simulink model "DualStreamSSR"  (R2020b)
(part 3 of 5)

  filter30 : ModelComposer/AIE Class Kernel  KernelAllAttrs=|  PortNames={'sin1'; 'sin2'; 'cout'}  PortSerializedTypes={'{Q2{P{Tinput_stream{1{t{Scint16}}}}}}'; '{Q2{P{Tinput_stream{1{t{Scint16}}}}}}'; '{P{Toutput_stream{1{t{Scacc48_t}}}}}'}  PortWindowSizes={0.000000000000000000e+00; 0.000000000000000000e+00; 0.000000000000000000e+00}  PortWindowMargins={0.000000000000000000e+00; 0.000000000000000000e+00; 0.000000000000000000e+00}  PortSynchronicities={'auto'; 'auto'; 'auto'}  PortSignalSizes={0.000000000000000000e+00; 0.000000000000000000e+00; 8.000000000000000000e+00}  ClassTemplateSpecKind=implicit  ClassTemplateParamNames={'NSamples'; 'ShiftAcc'; 'DiscardSample'; 'SwapRead'}  ClassTemplateParamKinds={'nontype'; 'nontype'; 'nontype'; 'nontype'}  ClassTemplateParamTypes={'int'; 'int'; 'bool'; 'bool'}  ClassTemplateParamValues={'512', '15', '0', '0'}  ClassCtorParamNames={'taps'}  ClassCtorParamSerializedTypes={'{R{Q1{C{Scint16}4}}}'}  ClassCtorParamValues={'[-121-233i 237-96i 1454+497i 14+121i]'}  ClassIndex=1  ClassCtorIndex=1  ClassTabVisible=on  ClassTemplateParamsVisible=on  ClassCtorDeclVisible=on  ClassCtorParamsVisible=on  FunctionTabVisible=on  FunctionDecl=|  PortAttrs={ 'input', 'sin1', 'input_stream_cint16 * restrict', '', '', '', ''; 'input', 'sin2', 'input_stream_cint16 * restrict', '', '', '', ''; 'output', 'cout', 'output_stream< cacc48_t > *', '', '', '', 'OUTPUT_SIZE' }  PortAttrsEnables={'off', 'off', 'off', 'off', 'off', 'off', 'off';'off', 'off', 'off', 'off', 'off', 'off', 'off';'off', 'off', 'off', 'off', 'off', 'off', 'on'}  SampleTime=-1  ClassDeclTypeOptions=|  ClassDecl=|  ClassTemplateParams={ 'NSamples', 'int', 'BURST_LENGTH'; 'ShiftAcc', 'int', 'SHIFT_ACC'; 'DiscardSample', 'bool', 'FALSE'; 'SwapRead', 'bool', 'FALSE' }  ClassTemplateParamsEnables={'off', 'off', 'on';'off', 'off', 'on';'off', 'off', 'on';'off', 'off', 'on'}  ClassCtorDeclTypeOptions=C[1 1]@t51@FIR_MultiKernel_cout(cint16 const ( & taps ) [ 4 ])  ClassCtorDecl=FIR_MultiKernel_cout(cint16 const ( & taps ) [ 4 ])  ClassCtorParams={ 'taps', 'cint16 const ( &) [ 4 ]', 'phi_4' }  KernelHeaderFile=FirDoubleStream.h  KernelClassName=DoubleStream::FIR_MultiKernel_cout  KernelFunction=filter  KernelSourceFile=FirDoubleStream.cpp  KernelSearchPaths={'$SRC/aie_kernels'}  PreProcOptions={}  CoreRuntimeRatio=0.9  KernelLocSpec=off  ColRowLocation=[0 0]  blockJsonConstraints="[{\"type\":\"constraint\",\"constraintType\":\"coreUtilization\",\"sid\":\"49\",\"lhs\":{\"type\":\"runtimeRatio\",\"args\":{\"type\":\"kernel\",\"name\":\"DualStreamSSR_1/Subsystem/filter30\",\"sid\":\"49\"}},\"rhs\":{\"type\":\"evaluable\",\"expr\":\"0.9\",\"value\":0.9},\"equality\":true},{\"type\":\"constraint\",\"constraintType\":\"location_kernel\",\"sid\":\"49\",\"lhs\":{\"type\":\"location\",\"templParam\":\"kernel\",\"args\":{\"type\":\"kernel\",\"name\":\"DualStreamSSR_1/Subsystem/filter30\",\"sid\":\"49\"}},\"rhs\":{\"type\":\"tile\",\"args\":[{\"type\":\"evaluable\",\"expr\":\"30\",\"value\":30},{\"type\":\"evaluable\",\"expr\":\"3\",\"value\":3}]},\"equality\":true}]"  deprecateConstraints=1
      KernelAllAttrs=|
      | s[12;12;9;9;19;14;21;23;24;21;12;24;26;26;26;27;28;9;21;23;23;23;24;25;14;19;19;29]@FunctionNameDeclFileNamePortNamesPortTypesPortSerializedTypesPortDirectionsPortWindowSizeEnablesPortWindowMarginEnablesPortSynchronicityEnablesPortSignalSizeEnablesFunctionDeclFunctionTemplateSpecKindFunctionTemplateParamNamesFunctionTemplateParamKindsFunctionTemplateParamTypesFunctionTemplateParamValuesFunctionTemplateParamEnablesClassDeclClassTemplateSpecKindClassTemplateParamNamesClassTemplateParamKindsClassTemplateParamTypesClassTemplateParamValuesClassTemplateParamEnablesClassCtorDeclsClassCtorParamNamesClassCtorParamTypesClassCtorParamSerializedTypes[1 1]@C[28 1]@t6@filtert42@../../../aie/aie_kernels/FirDoubleStream.hC[3 1]@t4@sin1t4@sin2t4@coutC[3 1]@t30@input_stream_cint16 * restrictt30@input_stream_cint16 * restrictt27@output_stream< cacc48_t > *C[3 1]@t37@{Q2{P{Tinput_stream{1{t{Scint16}}}}}}t37@{Q2{P{Tinput_stream{1{t{Scint16}}}}}}t36@{P{Toutput_stream{1{t{Scacc48_t}}}}}C[3 1]@t5@inputt5@inputt6@outputC[3 1]@l0@l0@l0@C[3 1]@l0@l0@l0@C[3 1]@l0@l0@l0@C[3 1]@l0@l0@l1@t246@namespace DoubleStream {
      | template < int NSamples, int ShiftAcc, bool DiscardSample, bool SwapRead > 
      | void FIR_MultiKernel_cout::
      | filter(input_stream_cint16 * restrict sin1, input_stream_cint16 * restrict sin2, output_stream< cacc48_t > * cout);
      | }t4@nonee[0 1]@e[0 1]@e[0 1]@e[0 1]@e[0 1]@t129@namespace DoubleStream {
      | template < int NSamples, int ShiftAcc, bool DiscardSample, bool SwapRead > class FIR_MultiKernel_cout;
      | }t8@implicitC[4 1]@t8@NSamplest8@ShiftAcct13@DiscardSamplet8@SwapReadC[4 1]@t7@nontypet7@nontypet7@nontypet7@nontypeC[4 1]@t3@intt3@intt4@boolt4@boolC[4 1]@nnnnC[4 1]@l1@l1@l1@l1@C[1 1]@t51@FIR_MultiKernel_cout(cint16 const ( & taps ) [ 4 ])C[1 1]@C[1 1]@t4@tapsC[1 1]@C[1 1]@t23@cint16 const ( &) [ 4 ]C[1 1]@C[1 1]@t20@{R{Q1{C{Scint16}4}}}
      FunctionDecl=|
      | namespace DoubleStream {
      | template < int NSamples, int ShiftAcc, bool DiscardSample, bool SwapRead > 
      | void FIR_MultiKernel_cout::
      | filter(input_stream_cint16 * restrict sin1, input_stream_cint16 * restrict sin2, output_stream< cacc48_t > * cout);
      | }
      ClassDeclTypeOptions=|
      | C[1 1]@t129@namespace DoubleStream {
      | template < int NSamples, int ShiftAcc, bool DiscardSample, bool SwapRead > class FIR_MultiKernel_cout;
      | }
      ClassDecl=|
      | namespace DoubleStream {
      | template < int NSamples, int ShiftAcc, bool DiscardSample, bool SwapRead > class FIR_MultiKernel_cout;
      | }
  filter31 : ModelComposer/AIE Class Kernel  KernelAllAttrs=|  PortNames={'sin1'; 'sin2'; 'cin'; 'cout'}  PortSerializedTypes={'{Q2{P{Tinput_stream{1{t{Scint16}}}}}}'; '{Q2{P{Tinput_stream{1{t{Scint16}}}}}}'; '{P{Tinput_stream{1{t{Scacc48_t}}}}}'; '{P{Toutput_stream{1{t{Scacc48_t}}}}}'}  PortWindowSizes={0.000000000000000000e+00; 0.000000000000000000e+00; 0.000000000000000000e+00; 0.000000000000000000e+00}  PortWindowMargins={0.000000000000000000e+00; 0.000000000000000000e+00; 0.000000000000000000e+00; 0.000000000000000000e+00}  PortSynchronicities={'auto'; 'auto'; 'auto'; 'auto'}  PortSignalSizes={0.000000000000000000e+00; 0.000000000000000000e+00; 0.000000000000000000e+00; 8.000000000000000000e+00}  ClassTemplateSpecKind=implicit  ClassTemplateParamNames={'NSamples'; 'ShiftAcc'; 'DiscardSample'; 'SwapRead'}  ClassTemplateParamKinds={'nontype'; 'nontype'; 'nontype'; 'nontype'}  ClassTemplateParamTypes={'int'; 'int'; 'bool'; 'bool'}  ClassTemplateParamValues={'512', '15', '0', '0'}  ClassCtorParamNames={'taps'}  ClassCtorParamSerializedTypes={'{R{Q1{C{Scint16}4}}}'}  ClassCtorParamValues={'[14-121i 1454-497i 237+96i -121+233i]'}  ClassIndex=1  ClassCtorIndex=1  ClassTabVisible=on  ClassTemplateParamsVisible=on  ClassCtorDeclVisible=on  ClassCtorParamsVisible=on  FunctionTabVisible=on  FunctionDecl=|  PortAttrs={ 'input', 'sin1', 'input_stream_cint16 * restrict', '', '', '', ''; 'input', 'sin2', 'input_stream_cint16 * restrict', '', '', '', ''; 'input', 'cin', 'input_stream< cacc48_t > *', '', '', '', ''; 'output', 'cout', 'output_stream< cacc48_t > *', '', '', '', 'OUTPUT_SIZE' }  PortAttrsEnables={'off', 'off', 'off', 'off', 'off', 'off', 'off';'off', 'off', 'off', 'off', 'off', 'off', 'off';'off', 'off', 'off', 'off', 'off', 'off', 'off';'off', 'off', 'off', 'off', 'off', 'off', 'on'}  SampleTime=-1  ClassDeclTypeOptions=|  ClassDecl=|  ClassTemplateParams={ 'NSamples', 'int', 'BURST_LENGTH'; 'ShiftAcc', 'int', 'SHIFT_ACC'; 'DiscardSample', 'bool', 'FALSE'; 'SwapRead', 'bool', 'FALSE' }  ClassTemplateParamsEnables={'off', 'off', 'on';'off', 'off', 'on';'off', 'off', 'on';'off', 'off', 'on'}  ClassCtorDeclTypeOptions=C[1 1]@t54@FIR_MultiKernel_cincout(cint16 const ( & taps ) [ 4 ])  ClassCtorDecl=FIR_MultiKernel_cincout(cint16 const ( & taps ) [ 4 ])  ClassCtorParams={ 'taps', 'cint16 const ( &) [ 4 ]', 'phi_3' }  KernelHeaderFile=FirDoubleStream.h  KernelClassName=DoubleStream::FIR_MultiKernel_cincout  KernelFunction=filter  KernelSourceFile=FirDoubleStream.cpp  KernelSearchPaths={'$SRC/aie_kernels'}  PreProcOptions={}  CoreRuntimeRatio=0.9  KernelLocSpec=off  ColRowLocation=[0 0]  blockJsonConstraints="{\"type\":\"constraint\",\"constraintType\":\"coreUtilization\",\"sid\":\"41\",\"lhs\":{\"type\":\"runtimeRatio\",\"args\":{\"type\":\"kernel\",\"name\":\"DualStreamSSR_1/Subsystem/filter22\",\"sid\":\"41\"}},\"rhs\":{\"type\":\"evaluable\",\"expr\":\"0.9\",\"value\":0.9},\"equality\":true}"  deprecateConstraints=1
      KernelAllAttrs=|
      | s[12;12;9;9;19;14;21;23;24;21;12;24;26;26;26;27;28;9;21;23;23;23;24;25;14;19;19;29]@FunctionNameDeclFileNamePortNamesPortTypesPortSerializedTypesPortDirectionsPortWindowSizeEnablesPortWindowMarginEnablesPortSynchronicityEnablesPortSignalSizeEnablesFunctionDeclFunctionTemplateSpecKindFunctionTemplateParamNamesFunctionTemplateParamKindsFunctionTemplateParamTypesFunctionTemplateParamValuesFunctionTemplateParamEnablesClassDeclClassTemplateSpecKindClassTemplateParamNamesClassTemplateParamKindsClassTemplateParamTypesClassTemplateParamValuesClassTemplateParamEnablesClassCtorDeclsClassCtorParamNamesClassCtorParamTypesClassCtorParamSerializedTypes[1 1]@C[28 1]@t6@filtert42@../../../aie/aie_kernels/FirDoubleStream.hC[4 1]@t4@sin1t4@sin2t3@cint4@coutC[4 1]@t30@input_stream_cint16 * restrictt30@input_stream_cint16 * restrictt26@input_stream< cacc48_t > *t27@output_stream< cacc48_t > *C[4 1]@t37@{Q2{P{Tinput_stream{1{t{Scint16}}}}}}t37@{Q2{P{Tinput_stream{1{t{Scint16}}}}}}t35@{P{Tinput_stream{1{t{Scacc48_t}}}}}t36@{P{Toutput_stream{1{t{Scacc48_t}}}}}C[4 1]@t5@inputt5@inputt5@inputt6@outputC[4 1]@l0@l0@l0@l0@C[4 1]@l0@l0@l0@l0@C[4 1]@l0@l0@l0@l0@C[4 1]@l0@l0@l0@l1@t281@namespace DoubleStream {
      | template < int NSamples, int ShiftAcc, bool DiscardSample, bool SwapRead > 
      | void FIR_MultiKernel_cincout::
      | filter(input_stream_cint16 * restrict sin1, input_stream_cint16 * restrict sin2, input_stream< cacc48_t > * cin, output_stream< cacc48_t > * cout);
      | }t4@nonee[0 1]@e[0 1]@e[0 1]@e[0 1]@e[0 1]@t132@namespace DoubleStream {
      | template < int NSamples, int ShiftAcc, bool DiscardSample, bool SwapRead > class FIR_MultiKernel_cincout;
      | }t8@implicitC[4 1]@t8@NSamplest8@ShiftAcct13@DiscardSamplet8@SwapReadC[4 1]@t7@nontypet7@nontypet7@nontypet7@nontypeC[4 1]@t3@intt3@intt4@boolt4@boolC[4 1]@nnnnC[4 1]@l1@l1@l1@l1@C[1 1]@t54@FIR_MultiKernel_cincout(cint16 const ( & taps ) [ 4 ])C[1 1]@C[1 1]@t4@tapsC[1 1]@C[1 1]@t23@cint16 const ( &) [ 4 ]C[1 1]@C[1 1]@t20@{R{Q1{C{Scint16}4}}}
      FunctionDecl=|
      | namespace DoubleStream {
      | template < int NSamples, int ShiftAcc, bool DiscardSample, bool SwapRead > 
      | void FIR_MultiKernel_cincout::
      | filter(input_stream_cint16 * restrict sin1, input_stream_cint16 * restrict sin2, input_stream< cacc48_t > * cin, output_stream< cacc48_t > * cout);
      | }
      ClassDeclTypeOptions=|
      | C[1 1]@t132@namespace DoubleStream {
      | template < int NSamples, int ShiftAcc, bool DiscardSample, bool SwapRead > class FIR_MultiKernel_cincout;
      | }
      ClassDecl=|
      | namespace DoubleStream {
      | template < int NSamples, int ShiftAcc, bool DiscardSample, bool SwapRead > class FIR_MultiKernel_cincout;
      | }
  filter32 : ModelComposer/AIE Class Kernel  KernelAllAttrs=|  PortNames={'sin1'; 'sin2'; 'cout'}  PortSerializedTypes={'{Q2{P{Tinput_stream{1{t{Scint16}}}}}}'; '{Q2{P{Tinput_stream{1{t{Scint16}}}}}}'; '{P{Toutput_stream{1{t{Scacc48_t}}}}}'}  PortWindowSizes={0.000000000000000000e+00; 0.000000000000000000e+00; 0.000000000000000000e+00}  PortWindowMargins={0.000000000000000000e+00; 0.000000000000000000e+00; 0.000000000000000000e+00}  PortSynchronicities={'auto'; 'auto'; 'auto'}  PortSignalSizes={0.000000000000000000e+00; 0.000000000000000000e+00; 8.000000000000000000e+00}  ClassTemplateSpecKind=implicit  ClassTemplateParamNames={'NSamples'; 'ShiftAcc'; 'DiscardSample'; 'SwapRead'}  ClassTemplateParamKinds={'nontype'; 'nontype'; 'nontype'; 'nontype'}  ClassTemplateParamTypes={'int'; 'int'; 'bool'; 'bool'}  ClassTemplateParamValues={'512', '15', '1', '0'}  ClassCtorParamNames={'taps'}  ClassCtorParamSerializedTypes={'{R{Q1{C{Scint16}4}}}'}  ClassCtorParamValues={'[-121-233i 237-96i 1454+497i 14+121i]'}  ClassIndex=1  ClassCtorIndex=1  ClassTabVisible=on  ClassTemplateParamsVisible=on  ClassCtorDeclVisible=on  ClassCtorParamsVisible=on  FunctionTabVisible=on  FunctionDecl=|  PortAttrs={ 'input', 'sin1', 'input_stream_cint16 * restrict', '', '', '', ''; 'input', 'sin2', 'input_stream_cint16 * restrict', '', '', '', ''; 'output', 'cout', 'output_stream< cacc48_t > *', '', '', '', 'OUTPUT_SIZE' }  PortAttrsEnables={'off', 'off', 'off', 'off', 'off', 'off', 'off';'off', 'off', 'off', 'off', 'off', 'off', 'off';'off', 'off', 'off', 'off', 'off', 'off', 'on'}  SampleTime=-1  ClassDeclTypeOptions=|  ClassDecl=|  ClassTemplateParams={ 'NSamples', 'int', 'BURST_LENGTH'; 'ShiftAcc', 'int', 'SHIFT_ACC'; 'DiscardSample', 'bool', 'TRUE'; 'SwapRead', 'bool', 'FALSE' }  ClassTemplateParamsEnables={'off', 'off', 'on';'off', 'off', 'on';'off', 'off', 'on';'off', 'off', 'on'}  ClassCtorDeclTypeOptions=C[1 1]@t51@FIR_MultiKernel_cout(cint16 const ( & taps ) [ 4 ])  ClassCtorDecl=FIR_MultiKernel_cout(cint16 const ( & taps ) [ 4 ])  ClassCtorParams={ 'taps', 'cint16 const ( &) [ 4 ]', 'phi_4' }  KernelHeaderFile=FirDoubleStream.h  KernelClassName=DoubleStream::FIR_MultiKernel_cout  KernelFunction=filter  KernelSourceFile=FirDoubleStream.cpp  KernelSearchPaths={'$SRC/aie_kernels'}  PreProcOptions={}  CoreRuntimeRatio=0.9  KernelLocSpec=off  ColRowLocation=[0 0]  blockJsonConstraints="[{\"type\":\"constraint\",\"constraintType\":\"coreUtilization\",\"sid\":\"51\",\"lhs\":{\"type\":\"runtimeRatio\",\"args\":{\"type\":\"kernel\",\"name\":\"DualStreamSSR_1/Subsystem/filter32\",\"sid\":\"51\"}},\"rhs\":{\"type\":\"evaluable\",\"expr\":\"0.9\",\"value\":0.9},\"equality\":true},{\"type\":\"constraint\",\"constraintType\":\"location_kernel\",\"sid\":\"51\",\"lhs\":{\"type\":\"location\",\"templParam\":\"kernel\",\"args\":{\"type\":\"kernel\",\"name\":\"DualStreamSSR_1/Subsystem/filter32\",\"sid\":\"51\"}},\"rhs\":{\"type\":\"tile\",\"args\":[{\"type\":\"evaluable\",\"expr\":\"23\",\"value\":23},{\"type\":\"evaluable\",\"expr\":\"4\",\"value\":4}]},\"equality\":true}]"  deprecateConstraints=1
      KernelAllAttrs=|
      | s[12;12;9;9;19;14;21;23;24;21;12;24;26;26;26;27;28;9;21;23;23;23;24;25;14;19;19;29]@FunctionNameDeclFileNamePortNamesPortTypesPortSerializedTypesPortDirectionsPortWindowSizeEnablesPortWindowMarginEnablesPortSynchronicityEnablesPortSignalSizeEnablesFunctionDeclFunctionTemplateSpecKindFunctionTemplateParamNamesFunctionTemplateParamKindsFunctionTemplateParamTypesFunctionTemplateParamValuesFunctionTemplateParamEnablesClassDeclClassTemplateSpecKindClassTemplateParamNamesClassTemplateParamKindsClassTemplateParamTypesClassTemplateParamValuesClassTemplateParamEnablesClassCtorDeclsClassCtorParamNamesClassCtorParamTypesClassCtorParamSerializedTypes[1 1]@C[28 1]@t6@filtert42@../../../aie/aie_kernels/FirDoubleStream.hC[3 1]@t4@sin1t4@sin2t4@coutC[3 1]@t30@input_stream_cint16 * restrictt30@input_stream_cint16 * restrictt27@output_stream< cacc48_t > *C[3 1]@t37@{Q2{P{Tinput_stream{1{t{Scint16}}}}}}t37@{Q2{P{Tinput_stream{1{t{Scint16}}}}}}t36@{P{Toutput_stream{1{t{Scacc48_t}}}}}C[3 1]@t5@inputt5@inputt6@outputC[3 1]@l0@l0@l0@C[3 1]@l0@l0@l0@C[3 1]@l0@l0@l0@C[3 1]@l0@l0@l1@t246@namespace DoubleStream {
      | template < int NSamples, int ShiftAcc, bool DiscardSample, bool SwapRead > 
      | void FIR_MultiKernel_cout::
      | filter(input_stream_cint16 * restrict sin1, input_stream_cint16 * restrict sin2, output_stream< cacc48_t > * cout);
      | }t4@nonee[0 1]@e[0 1]@e[0 1]@e[0 1]@e[0 1]@t129@namespace DoubleStream {
      | template < int NSamples, int ShiftAcc, bool DiscardSample, bool SwapRead > class FIR_MultiKernel_cout;
      | }t8@implicitC[4 1]@t8@NSamplest8@ShiftAcct13@DiscardSamplet8@SwapReadC[4 1]@t7@nontypet7@nontypet7@nontypet7@nontypeC[4 1]@t3@intt3@intt4@boolt4@boolC[4 1]@nnnnC[4 1]@l1@l1@l1@l1@C[1 1]@t51@FIR_MultiKernel_cout(cint16 const ( & taps ) [ 4 ])C[1 1]@C[1 1]@t4@tapsC[1 1]@C[1 1]@t23@cint16 const ( &) [ 4 ]C[1 1]@C[1 1]@t20@{R{Q1{C{Scint16}4}}}
      FunctionDecl=|
      | namespace DoubleStream {
      | template < int NSamples, int ShiftAcc, bool DiscardSample, bool SwapRead > 
      | void FIR_MultiKernel_cout::
      | filter(input_stream_cint16 * restrict sin1, input_stream_cint16 * restrict sin2, output_stream< cacc48_t > * cout);
      | }
      ClassDeclTypeOptions=|
      | C[1 1]@t129@namespace DoubleStream {
      | template < int NSamples, int ShiftAcc, bool DiscardSample, bool SwapRead > class FIR_MultiKernel_cout;
      | }
      ClassDecl=|
      | namespace DoubleStream {
      | template < int NSamples, int ShiftAcc, bool DiscardSample, bool SwapRead > class FIR_MultiKernel_cout;
      | }
  filter33 : ModelComposer/AIE Class Kernel  KernelAllAttrs=|  PortNames={'sin1'; 'sin2'; 'cin'; 'cout'}  PortSerializedTypes={'{Q2{P{Tinput_stream{1{t{Scint16}}}}}}'; '{Q2{P{Tinput_stream{1{t{Scint16}}}}}}'; '{P{Tinput_stream{1{t{Scacc48_t}}}}}'; '{P{Toutput_stream{1{t{Scacc48_t}}}}}'}  PortWindowSizes={0.000000000000000000e+00; 0.000000000000000000e+00; 0.000000000000000000e+00; 0.000000000000000000e+00}  PortWindowMargins={0.000000000000000000e+00; 0.000000000000000000e+00; 0.000000000000000000e+00; 0.000000000000000000e+00}  PortSynchronicities={'auto'; 'auto'; 'auto'; 'auto'}  PortSignalSizes={0.000000000000000000e+00; 0.000000000000000000e+00; 0.000000000000000000e+00; 8.000000000000000000e+00}  ClassTemplateSpecKind=implicit  ClassTemplateParamNames={'NSamples'; 'ShiftAcc'; 'DiscardSample'; 'SwapRead'}  ClassTemplateParamKinds={'nontype'; 'nontype'; 'nontype'; 'nontype'}  ClassTemplateParamTypes={'int'; 'int'; 'bool'; 'bool'}  ClassTemplateParamValues={'512', '15', '1', '0'}  ClassCtorParamNames={'taps'}  ClassCtorParamSerializedTypes={'{R{Q1{C{Scint16}4}}}'}  ClassCtorParamValues={'[-160-111i 248+2878i 1183-239i -21-26i]'}  ClassIndex=1  ClassCtorIndex=1  ClassTabVisible=on  ClassTemplateParamsVisible=on  ClassCtorDeclVisible=on  ClassCtorParamsVisible=on  FunctionTabVisible=on  FunctionDecl=|  PortAttrs={ 'input', 'sin1', 'input_stream_cint16 * restrict', '', '', '', ''; 'input', 'sin2', 'input_stream_cint16 * restrict', '', '', '', ''; 'input', 'cin', 'input_stream< cacc48_t > *', '', '', '', ''; 'output', 'cout', 'output_stream< cacc48_t > *', '', '', '', 'OUTPUT_SIZE' }  PortAttrsEnables={'off', 'off', 'off', 'off', 'off', 'off', 'off';'off', 'off', 'off', 'off', 'off', 'off', 'off';'off', 'off', 'off', 'off', 'off', 'off', 'off';'off', 'off', 'off', 'off', 'off', 'off', 'on'}  SampleTime=-1  ClassDeclTypeOptions=|  ClassDecl=|  ClassTemplateParams={ 'NSamples', 'int', 'BURST_LENGTH'; 'ShiftAcc', 'int', 'SHIFT_ACC'; 'DiscardSample', 'bool', 'TRUE'; 'SwapRead', 'bool', 'FALSE' }  ClassTemplateParamsEnables={'off', 'off', 'on';'off', 'off', 'on';'off', 'off', 'on';'off', 'off', 'on'}  ClassCtorDeclTypeOptions=C[1 1]@t54@FIR_MultiKernel_cincout(cint16 const ( & taps ) [ 4 ])  ClassCtorDecl=FIR_MultiKernel_cincout(cint16 const ( & taps ) [ 4 ])  ClassCtorParams={ 'taps', 'cint16 const ( &) [ 4 ]', 'phi_5' }  KernelHeaderFile=FirDoubleStream.h  KernelClassName=DoubleStream::FIR_MultiKernel_cincout  KernelFunction=filter  KernelSourceFile=FirDoubleStream.cpp  KernelSearchPaths={'$SRC/aie_kernels'}  PreProcOptions={}  CoreRuntimeRatio=0.9  KernelLocSpec=off  ColRowLocation=[0 0]  blockJsonConstraints="{\"type\":\"constraint\",\"constraintType\":\"coreUtilization\",\"sid\":\"52\",\"lhs\":{\"type\":\"runtimeRatio\",\"args\":{\"type\":\"kernel\",\"name\":\"DualStreamSSR_1/Subsystem/filter33\",\"sid\":\"52\"}},\"rhs\":{\"type\":\"evaluable\",\"expr\":\"0.9\",\"value\":0.9},\"equality\":true}"  deprecateConstraints=1
      KernelAllAttrs=|
      | s[12;12;9;9;19;14;21;23;24;21;12;24;26;26;26;27;28;9;21;23;23;23;24;25;14;19;19;29]@FunctionNameDeclFileNamePortNamesPortTypesPortSerializedTypesPortDirectionsPortWindowSizeEnablesPortWindowMarginEnablesPortSynchronicityEnablesPortSignalSizeEnablesFunctionDeclFunctionTemplateSpecKindFunctionTemplateParamNamesFunctionTemplateParamKindsFunctionTemplateParamTypesFunctionTemplateParamValuesFunctionTemplateParamEnablesClassDeclClassTemplateSpecKindClassTemplateParamNamesClassTemplateParamKindsClassTemplateParamTypesClassTemplateParamValuesClassTemplateParamEnablesClassCtorDeclsClassCtorParamNamesClassCtorParamTypesClassCtorParamSerializedTypes[1 1]@C[28 1]@t6@filtert42@../../../aie/aie_kernels/FirDoubleStream.hC[4 1]@t4@sin1t4@sin2t3@cint4@coutC[4 1]@t30@input_stream_cint16 * restrictt30@input_stream_cint16 * restrictt26@input_stream< cacc48_t > *t27@output_stream< cacc48_t > *C[4 1]@t37@{Q2{P{Tinput_stream{1{t{Scint16}}}}}}t37@{Q2{P{Tinput_stream{1{t{Scint16}}}}}}t35@{P{Tinput_stream{1{t{Scacc48_t}}}}}t36@{P{Toutput_stream{1{t{Scacc48_t}}}}}C[4 1]@t5@inputt5@inputt5@inputt6@outputC[4 1]@l0@l0@l0@l0@C[4 1]@l0@l0@l0@l0@C[4 1]@l0@l0@l0@l0@C[4 1]@l0@l0@l0@l1@t281@namespace DoubleStream {
      | template < int NSamples, int ShiftAcc, bool DiscardSample, bool SwapRead > 
      | void FIR_MultiKernel_cincout::
      | filter(input_stream_cint16 * restrict sin1, input_stream_cint16 * restrict sin2, input_stream< cacc48_t > * cin, output_stream< cacc48_t > * cout);
      | }t4@nonee[0 1]@e[0 1]@e[0 1]@e[0 1]@e[0 1]@t132@namespace DoubleStream {
      | template < int NSamples, int ShiftAcc, bool DiscardSample, bool SwapRead > class FIR_MultiKernel_cincout;
      | }t8@implicitC[4 1]@t8@NSamplest8@ShiftAcct13@DiscardSamplet8@SwapReadC[4 1]@t7@nontypet7@nontypet7@nontypet7@nontypeC[4 1]@t3@intt3@intt4@boolt4@boolC[4 1]@nnnnC[4 1]@l1@l1@l1@l1@C[1 1]@t54@FIR_MultiKernel_cincout(cint16 const ( & taps ) [ 4 ])C[1 1]@C[1 1]@t4@tapsC[1 1]@C[1 1]@t23@cint16 const ( &) [ 4 ]C[1 1]@C[1 1]@t20@{R{Q1{C{Scint16}4}}}
      FunctionDecl=|
      | namespace DoubleStream {
      | template < int NSamples, int ShiftAcc, bool DiscardSample, bool SwapRead > 
      | void FIR_MultiKernel_cincout::
      | filter(input_stream_cint16 * restrict sin1, input_stream_cint16 * restrict sin2, input_stream< cacc48_t > * cin, output_stream< cacc48_t > * cout);
      | }
      ClassDeclTypeOptions=|
      | C[1 1]@t132@namespace DoubleStream {
      | template < int NSamples, int ShiftAcc, bool DiscardSample, bool SwapRead > class FIR_MultiKernel_cincout;
      | }
      ClassDecl=|
      | namespace DoubleStream {
      | template < int NSamples, int ShiftAcc, bool DiscardSample, bool SwapRead > class FIR_MultiKernel_cincout;
      | }
  filter34 : ModelComposer/AIE Class Kernel  KernelAllAttrs=|  PortNames={'sin1'; 'sin2'; 'cin'; 'cout'}  PortSerializedTypes={'{Q2{P{Tinput_stream{1{t{Scint16}}}}}}'; '{Q2{P{Tinput_stream{1{t{Scint16}}}}}}'; '{P{Tinput_stream{1{t{Scacc48_t}}}}}'; '{P{Toutput_stream{1{t{Scacc48_t}}}}}'}  PortWindowSizes={0.000000000000000000e+00; 0.000000000000000000e+00; 0.000000000000000000e+00; 0.000000000000000000e+00}  PortWindowMargins={0.000000000000000000e+00; 0.000000000000000000e+00; 0.000000000000000000e+00; 0.000000000000000000e+00}  PortSynchronicities={'auto'; 'auto'; 'auto'; 'auto'}  PortSignalSizes={0.000000000000000000e+00; 0.000000000000000000e+00; 0.000000000000000000e+00; 8.000000000000000000e+00}  ClassTemplateSpecKind=implicit  ClassTemplateParamNames={'NSamples'; 'ShiftAcc'; 'DiscardSample'; 'SwapRead'}  ClassTemplateParamKinds={'nontype'; 'nontype'; 'nontype'; 'nontype'}  ClassTemplateParamTypes={'int'; 'int'; 'bool'; 'bool'}  ClassTemplateParamValues={'512', '15', '1', '0'}  ClassCtorParamNames={'taps'}  ClassCtorParamSerializedTypes={'{R{Q1{C{Scint16}4}}}'}  ClassCtorParamValues={'[-160-111i 248+2878i 1183-239i -21-26i]'}  ClassIndex=1  ClassCtorIndex=1  ClassTabVisible=on  ClassTemplateParamsVisible=on  ClassCtorDeclVisible=on  ClassCtorParamsVisible=on  FunctionTabVisible=on  FunctionDecl=|  PortAttrs={ 'input', 'sin1', 'input_stream_cint16 * restrict', '', '', '', ''; 'input', 'sin2', 'input_stream_cint16 * restrict', '', '', '', ''; 'input', 'cin', 'input_stream< cacc48_t > *', '', '', '', ''; 'output', 'cout', 'output_stream< cacc48_t > *', '', '', '', 'OUTPUT_SIZE' }  PortAttrsEnables={'off', 'off', 'off', 'off', 'off', 'off', 'off';'off', 'off', 'off', 'off', 'off', 'off', 'off';'off', 'off', 'off', 'off', 'off', 'off', 'off';'off', 'off', 'off', 'off', 'off', 'off', 'on'}  SampleTime=-1  ClassDeclTypeOptions=|  ClassDecl=|  ClassTemplateParams={ 'NSamples', 'int', 'BURST_LENGTH'; 'ShiftAcc', 'int', 'SHIFT_ACC'; 'DiscardSample', 'bool', 'TRUE'; 'SwapRead', 'bool', 'FALSE' }  ClassTemplateParamsEnables={'off', 'off', 'on';'off', 'off', 'on';'off', 'off', 'on';'off', 'off', 'on'}  ClassCtorDeclTypeOptions=C[1 1]@t54@FIR_MultiKernel_cincout(cint16 const ( & taps ) [ 4 ])  ClassCtorDecl=FIR_MultiKernel_cincout(cint16 const ( & taps ) [ 4 ])  ClassCtorParams={ 'taps', 'cint16 const ( &) [ 4 ]', 'phi_5' }  KernelHeaderFile=FirDoubleStream.h  KernelClassName=DoubleStream::FIR_MultiKernel_cincout  KernelFunction=filter  KernelSourceFile=FirDoubleStream.cpp  KernelSearchPaths={'$SRC/aie_kernels'}  PreProcOptions={}  CoreRuntimeRatio=0.9  KernelLocSpec=off  ColRowLocation=[0 0]  blockJsonConstraints="{\"type\":\"constraint\",\"constraintType\":\"coreUtilization\",\"sid\":\"57\",\"lhs\":{\"type\":\"runtimeRatio\",\"args\":{\"type\":\"kernel\",\"name\":\"DualStreamSSR_1/Subsystem/filter38\",\"sid\":\"57\"}},\"rhs\":{\"type\":\"evaluable\",\"expr\":\"0.9\",\"value\":0.9},\"equality\":true}"  deprecateConstraints=1
      KernelAllAttrs=|
      | s[12;12;9;9;19;14;21;23;24;21;12;24;26;26;26;27;28;9;21;23;23;23;24;25;14;19;19;29]@FunctionNameDeclFileNamePortNamesPortTypesPortSerializedTypesPortDirectionsPortWindowSizeEnablesPortWindowMarginEnablesPortSynchronicityEnablesPortSignalSizeEnablesFunctionDeclFunctionTemplateSpecKindFunctionTemplateParamNamesFunctionTemplateParamKindsFunctionTemplateParamTypesFunctionTemplateParamValuesFunctionTemplateParamEnablesClassDeclClassTemplateSpecKindClassTemplateParamNamesClassTemplateParamKindsClassTemplateParamTypesClassTemplateParamValuesClassTemplateParamEnablesClassCtorDeclsClassCtorParamNamesClassCtorParamTypesClassCtorParamSerializedTypes[1 1]@C[28 1]@t6@filtert42@../../../aie/aie_kernels/FirDoubleStream.hC[4 1]@t4@sin1t4@sin2t3@cint4@coutC[4 1]@t30@input_stream_cint16 * restrictt30@input_stream_cint16 * restrictt26@input_stream< cacc48_t > *t27@output_stream< cacc48_t > *C[4 1]@t37@{Q2{P{Tinput_stream{1{t{Scint16}}}}}}t37@{Q2{P{Tinput_stream{1{t{Scint16}}}}}}t35@{P{Tinput_stream{1{t{Scacc48_t}}}}}t36@{P{Toutput_stream{1{t{Scacc48_t}}}}}C[4 1]@t5@inputt5@inputt5@inputt6@outputC[4 1]@l0@l0@l0@l0@C[4 1]@l0@l0@l0@l0@C[4 1]@l0@l0@l0@l0@C[4 1]@l0@l0@l0@l1@t281@namespace DoubleStream {
      | template < int NSamples, int ShiftAcc, bool DiscardSample, bool SwapRead > 
      | void FIR_MultiKernel_cincout::
      | filter(input_stream_cint16 * restrict sin1, input_stream_cint16 * restrict sin2, input_stream< cacc48_t > * cin, output_stream< cacc48_t > * cout);
      | }t4@nonee[0 1]@e[0 1]@e[0 1]@e[0 1]@e[0 1]@t132@namespace DoubleStream {
      | template < int NSamples, int ShiftAcc, bool DiscardSample, bool SwapRead > class FIR_MultiKernel_cincout;
      | }t8@implicitC[4 1]@t8@NSamplest8@ShiftAcct13@DiscardSamplet8@SwapReadC[4 1]@t7@nontypet7@nontypet7@nontypet7@nontypeC[4 1]@t3@intt3@intt4@boolt4@boolC[4 1]@nnnnC[4 1]@l1@l1@l1@l1@C[1 1]@t54@FIR_MultiKernel_cincout(cint16 const ( & taps ) [ 4 ])C[1 1]@C[1 1]@t4@tapsC[1 1]@C[1 1]@t23@cint16 const ( &) [ 4 ]C[1 1]@C[1 1]@t20@{R{Q1{C{Scint16}4}}}
      FunctionDecl=|
      | namespace DoubleStream {
      | template < int NSamples, int ShiftAcc, bool DiscardSample, bool SwapRead > 
      | void FIR_MultiKernel_cincout::
      | filter(input_stream_cint16 * restrict sin1, input_stream_cint16 * restrict sin2, input_stream< cacc48_t > * cin, output_stream< cacc48_t > * cout);
      | }
      ClassDeclTypeOptions=|
      | C[1 1]@t132@namespace DoubleStream {
      | template < int NSamples, int ShiftAcc, bool DiscardSample, bool SwapRead > class FIR_MultiKernel_cincout;
      | }
      ClassDecl=|
      | namespace DoubleStream {
      | template < int NSamples, int ShiftAcc, bool DiscardSample, bool SwapRead > class FIR_MultiKernel_cincout;
      | }
  filter35 : ModelComposer/AIE Class Kernel  KernelAllAttrs=|  PortNames={'sin1'; 'sin2'; 'cin'; 'cout'}  PortSerializedTypes={'{Q2{P{Tinput_stream{1{t{Scint16}}}}}}'; '{Q2{P{Tinput_stream{1{t{Scint16}}}}}}'; '{P{Tinput_stream{1{t{Scacc48_t}}}}}'; '{P{Toutput_stream{1{t{Scacc48_t}}}}}'}  PortWindowSizes={0.000000000000000000e+00; 0.000000000000000000e+00; 0.000000000000000000e+00; 0.000000000000000000e+00}  PortWindowMargins={0.000000000000000000e+00; 0.000000000000000000e+00; 0.000000000000000000e+00; 0.000000000000000000e+00}  PortSynchronicities={'auto'; 'auto'; 'auto'; 'auto'}  PortSignalSizes={0.000000000000000000e+00; 0.000000000000000000e+00; 0.000000000000000000e+00; 8.000000000000000000e+00}  ClassTemplateSpecKind=implicit  ClassTemplateParamNames={'NSamples'; 'ShiftAcc'; 'DiscardSample'; 'SwapRead'}  ClassTemplateParamKinds={'nontype'; 'nontype'; 'nontype'; 'nontype'}  ClassTemplateParamTypes={'int'; 'int'; 'bool'; 'bool'}  ClassTemplateParamValues={'512', '15', '1', '0'}  ClassCtorParamNames={'taps'}  ClassCtorParamSerializedTypes={'{R{Q1{C{Scint16}4}}}'}  ClassCtorParamValues={'[146-91i 4086+5221i 237-54i -83-21i]'}  ClassIndex=1  ClassCtorIndex=1  ClassTabVisible=on  ClassTemplateParamsVisible=on  ClassCtorDeclVisible=on  ClassCtorParamsVisible=on  FunctionTabVisible=on  FunctionDecl=|  PortAttrs={ 'input', 'sin1', 'input_stream_cint16 * restrict', '', '', '', ''; 'input', 'sin2', 'input_stream_cint16 * restrict', '', '', '', ''; 'input', 'cin', 'input_stream< cacc48_t > *', '', '', '', ''; 'output', 'cout', 'output_stream< cacc48_t > *', '', '', '', 'OUTPUT_SIZE' }  PortAttrsEnables={'off', 'off', 'off', 'off', 'off', 'off', 'off';'off', 'off', 'off', 'off', 'off', 'off', 'off';'off', 'off', 'off', 'off', 'off', 'off', 'off';'off', 'off', 'off', 'off', 'off', 'off', 'on'}  SampleTime=-1  ClassDeclTypeOptions=|  ClassDecl=|  ClassTemplateParams={ 'NSamples', 'int', 'BURST_LENGTH'; 'ShiftAcc', 'int', 'SHIFT_ACC'; 'DiscardSample', 'bool', 'TRUE'; 'SwapRead', 'bool', 'FALSE' }  ClassTemplateParamsEnables={'off', 'off', 'on';'off', 'off', 'on';'off', 'off', 'on';'off', 'off', 'on'}  ClassCtorDeclTypeOptions=C[1 1]@t54@FIR_MultiKernel_cincout(cint16 const ( & taps ) [ 4 ])  ClassCtorDecl=FIR_MultiKernel_cincout(cint16 const ( & taps ) [ 4 ])  ClassCtorParams={ 'taps', 'cint16 const ( &) [ 4 ]', 'phi_6' }  KernelHeaderFile=FirDoubleStream.h  KernelClassName=DoubleStream::FIR_MultiKernel_cincout  KernelFunction=filter  KernelSourceFile=FirDoubleStream.cpp  KernelSearchPaths={'$SRC/aie_kernels'}  PreProcOptions={}  CoreRuntimeRatio=0.9  KernelLocSpec=off  ColRowLocation=[0 0]  blockJsonConstraints="{\"type\":\"constraint\",\"constraintType\":\"coreUtilization\",\"sid\":\"57\",\"lhs\":{\"type\":\"runtimeRatio\",\"args\":{\"type\":\"kernel\",\"name\":\"DualStreamSSR_1/Subsystem/filter38\",\"sid\":\"57\"}},\"rhs\":{\"type\":\"evaluable\",\"expr\":\"0.9\",\"value\":0.9},\"equality\":true}"  deprecateConstraints=1
      KernelAllAttrs=|
      | s[12;12;9;9;19;14;21;23;24;21;12;24;26;26;26;27;28;9;21;23;23;23;24;25;14;19;19;29]@FunctionNameDeclFileNamePortNamesPortTypesPortSerializedTypesPortDirectionsPortWindowSizeEnablesPortWindowMarginEnablesPortSynchronicityEnablesPortSignalSizeEnablesFunctionDeclFunctionTemplateSpecKindFunctionTemplateParamNamesFunctionTemplateParamKindsFunctionTemplateParamTypesFunctionTemplateParamValuesFunctionTemplateParamEnablesClassDeclClassTemplateSpecKindClassTemplateParamNamesClassTemplateParamKindsClassTemplateParamTypesClassTemplateParamValuesClassTemplateParamEnablesClassCtorDeclsClassCtorParamNamesClassCtorParamTypesClassCtorParamSerializedTypes[1 1]@C[28 1]@t6@filtert42@../../../aie/aie_kernels/FirDoubleStream.hC[4 1]@t4@sin1t4@sin2t3@cint4@coutC[4 1]@t30@input_stream_cint16 * restrictt30@input_stream_cint16 * restrictt26@input_stream< cacc48_t > *t27@output_stream< cacc48_t > *C[4 1]@t37@{Q2{P{Tinput_stream{1{t{Scint16}}}}}}t37@{Q2{P{Tinput_stream{1{t{Scint16}}}}}}t35@{P{Tinput_stream{1{t{Scacc48_t}}}}}t36@{P{Toutput_stream{1{t{Scacc48_t}}}}}C[4 1]@t5@inputt5@inputt5@inputt6@outputC[4 1]@l0@l0@l0@l0@C[4 1]@l0@l0@l0@l0@C[4 1]@l0@l0@l0@l0@C[4 1]@l0@l0@l0@l1@t281@namespace DoubleStream {
      | template < int NSamples, int ShiftAcc, bool DiscardSample, bool SwapRead > 
      | void FIR_MultiKernel_cincout::
      | filter(input_stream_cint16 * restrict sin1, input_stream_cint16 * restrict sin2, input_stream< cacc48_t > * cin, output_stream< cacc48_t > * cout);
      | }t4@nonee[0 1]@e[0 1]@e[0 1]@e[0 1]@e[0 1]@t132@namespace DoubleStream {
      | template < int NSamples, int ShiftAcc, bool DiscardSample, bool SwapRead > class FIR_MultiKernel_cincout;
      | }t8@implicitC[4 1]@t8@NSamplest8@ShiftAcct13@DiscardSamplet8@SwapReadC[4 1]@t7@nontypet7@nontypet7@nontypet7@nontypeC[4 1]@t3@intt3@intt4@boolt4@boolC[4 1]@nnnnC[4 1]@l1@l1@l1@l1@C[1 1]@t54@FIR_MultiKernel_cincout(cint16 const ( & taps ) [ 4 ])C[1 1]@C[1 1]@t4@tapsC[1 1]@C[1 1]@t23@cint16 const ( &) [ 4 ]C[1 1]@C[1 1]@t20@{R{Q1{C{Scint16}4}}}
      FunctionDecl=|
      | namespace DoubleStream {
      | template < int NSamples, int ShiftAcc, bool DiscardSample, bool SwapRead > 
      | void FIR_MultiKernel_cincout::
      | filter(input_stream_cint16 * restrict sin1, input_stream_cint16 * restrict sin2, input_stream< cacc48_t > * cin, output_stream< cacc48_t > * cout);
      | }
      ClassDeclTypeOptions=|
      | C[1 1]@t132@namespace DoubleStream {
      | template < int NSamples, int ShiftAcc, bool DiscardSample, bool SwapRead > class FIR_MultiKernel_cincout;
      | }
      ClassDecl=|
      | namespace DoubleStream {
      | template < int NSamples, int ShiftAcc, bool DiscardSample, bool SwapRead > class FIR_MultiKernel_cincout;
      | }
  filter36 : ModelComposer/AIE Class Kernel  KernelAllAttrs=|  PortNames={'sin1'; 'sin2'; 'cin'; 'cout'}  PortSerializedTypes={'{Q2{P{Tinput_stream{1{t{Scint16}}}}}}'; '{Q2{P{Tinput_stream{1{t{Scint16}}}}}}'; '{P{Tinput_stream{1{t{Scacc48_t}}}}}'; '{P{Toutput_stream{1{t{Scacc48_t}}}}}'}  PortWindowSizes={0.000000000000000000e+00; 0.000000000000000000e+00; 0.000000000000000000e+00; 0.000000000000000000e+00}  PortWindowMargins={0.000000000000000000e+00; 0.000000000000000000e+00; 0.000000000000000000e+00; 0.000000000000000000e+00}  PortSynchronicities={'auto'; 'auto'; 'auto'; 'auto'}  PortSignalSizes={0.000000000000000000e+00; 0.000000000000000000e+00; 0.000000000000000000e+00; 8.000000000000000000e+00}  ClassTemplateSpecKind=implicit  ClassTemplateParamNames={'NSamples'; 'ShiftAcc'; 'DiscardSample'; 'SwapRead'}  ClassTemplateParamKinds={'nontype'; 'nontype'; 'nontype'; 'nontype'}  ClassTemplateParamTypes={'int'; 'int'; 'bool'; 'bool'}  ClassTemplateParamValues={'512', '15', '1', '0'}  ClassCtorParamNames={'taps'}  ClassCtorParamSerializedTypes={'{R{Q1{C{Scint16}4}}}'}  ClassCtorParamValues={'[342-439i 8773+2748i 102+525i -54+21i]'}  ClassIndex=1  ClassCtorIndex=1  ClassTabVisible=on  ClassTemplateParamsVisible=on  ClassCtorDeclVisible=on  ClassCtorParamsVisible=on  FunctionTabVisible=on  FunctionDecl=|  PortAttrs={ 'input', 'sin1', 'input_stream_cint16 * restrict', '', '', '', ''; 'input', 'sin2', 'input_stream_cint16 * restrict', '', '', '', ''; 'input', 'cin', 'input_stream< cacc48_t > *', '', '', '', ''; 'output', 'cout', 'output_stream< cacc48_t > *', '', '', '', 'OUTPUT_SIZE' }  PortAttrsEnables={'off', 'off', 'off', 'off', 'off', 'off', 'off';'off', 'off', 'off', 'off', 'off', 'off', 'off';'off', 'off', 'off', 'off', 'off', 'off', 'off';'off', 'off', 'off', 'off', 'off', 'off', 'on'}  SampleTime=-1  ClassDeclTypeOptions=|  ClassDecl=|  ClassTemplateParams={ 'NSamples', 'int', 'BURST_LENGTH'; 'ShiftAcc', 'int', 'SHIFT_ACC'; 'DiscardSample', 'bool', 'TRUE'; 'SwapRead', 'bool', 'FALSE' }  ClassTemplateParamsEnables={'off', 'off', 'on';'off', 'off', 'on';'off', 'off', 'on';'off', 'off', 'on'}  ClassCtorDeclTypeOptions=C[1 1]@t54@FIR_MultiKernel_cincout(cint16 const ( & taps ) [ 4 ])  ClassCtorDecl=FIR_MultiKernel_cincout(cint16 const ( & taps ) [ 4 ])  ClassCtorParams={ 'taps', 'cint16 const ( &) [ 4 ]', 'phi_7' }  KernelHeaderFile=FirDoubleStream.h  KernelClassName=DoubleStream::FIR_MultiKernel_cincout  KernelFunction=filter  KernelSourceFile=FirDoubleStream.cpp  KernelSearchPaths={'$SRC/aie_kernels'}  PreProcOptions={}  CoreRuntimeRatio=0.9  KernelLocSpec=off  ColRowLocation=[0 0]  blockJsonConstraints="{\"type\":\"constraint\",\"constraintType\":\"coreUtilization\",\"sid\":\"57\",\"lhs\":{\"type\":\"runtimeRatio\",\"args\":{\"type\":\"kernel\",\"name\":\"DualStreamSSR_1/Subsystem/filter38\",\"sid\":\"57\"}},\"rhs\":{\"type\":\"evaluable\",\"expr\":\"0.9\",\"value\":0.9},\"equality\":true}"  deprecateConstraints=1
      KernelAllAttrs=|
      | s[12;12;9;9;19;14;21;23;24;21;12;24;26;26;26;27;28;9;21;23;23;23;24;25;14;19;19;29]@FunctionNameDeclFileNamePortNamesPortTypesPortSerializedTypesPortDirectionsPortWindowSizeEnablesPortWindowMarginEnablesPortSynchronicityEnablesPortSignalSizeEnablesFunctionDeclFunctionTemplateSpecKindFunctionTemplateParamNamesFunctionTemplateParamKindsFunctionTemplateParamTypesFunctionTemplateParamValuesFunctionTemplateParamEnablesClassDeclClassTemplateSpecKindClassTemplateParamNamesClassTemplateParamKindsClassTemplateParamTypesClassTemplateParamValuesClassTemplateParamEnablesClassCtorDeclsClassCtorParamNamesClassCtorParamTypesClassCtorParamSerializedTypes[1 1]@C[28 1]@t6@filtert42@../../../aie/aie_kernels/FirDoubleStream.hC[4 1]@t4@sin1t4@sin2t3@cint4@coutC[4 1]@t30@input_stream_cint16 * restrictt30@input_stream_cint16 * restrictt26@input_stream< cacc48_t > *t27@output_stream< cacc48_t > *C[4 1]@t37@{Q2{P{Tinput_stream{1{t{Scint16}}}}}}t37@{Q2{P{Tinput_stream{1{t{Scint16}}}}}}t35@{P{Tinput_stream{1{t{Scacc48_t}}}}}t36@{P{Toutput_stream{1{t{Scacc48_t}}}}}C[4 1]@t5@inputt5@inputt5@inputt6@outputC[4 1]@l0@l0@l0@l0@C[4 1]@l0@l0@l0@l0@C[4 1]@l0@l0@l0@l0@C[4 1]@l0@l0@l0@l1@t281@namespace DoubleStream {
      | template < int NSamples, int ShiftAcc, bool DiscardSample, bool SwapRead > 
      | void FIR_MultiKernel_cincout::
      | filter(input_stream_cint16 * restrict sin1, input_stream_cint16 * restrict sin2, input_stream< cacc48_t > * cin, output_stream< cacc48_t > * cout);
      | }t4@nonee[0 1]@e[0 1]@e[0 1]@e[0 1]@e[0 1]@t132@namespace DoubleStream {
      | template < int NSamples, int ShiftAcc, bool DiscardSample, bool SwapRead > class FIR_MultiKernel_cincout;
      | }t8@implicitC[4 1]@t8@NSamplest8@ShiftAcct13@DiscardSamplet8@SwapReadC[4 1]@t7@nontypet7@nontypet7@nontypet7@nontypeC[4 1]@t3@intt3@intt4@boolt4@boolC[4 1]@nnnnC[4 1]@l1@l1@l1@l1@C[1 1]@t54@FIR_MultiKernel_cincout(cint16 const ( & taps ) [ 4 ])C[1 1]@C[1 1]@t4@tapsC[1 1]@C[1 1]@t23@cint16 const ( &) [ 4 ]C[1 1]@C[1 1]@t20@{R{Q1{C{Scint16}4}}}
      FunctionDecl=|
      | namespace DoubleStream {
      | template < int NSamples, int ShiftAcc, bool DiscardSample, bool SwapRead > 
      | void FIR_MultiKernel_cincout::
      | filter(input_stream_cint16 * restrict sin1, input_stream_cint16 * restrict sin2, input_stream< cacc48_t > * cin, output_stream< cacc48_t > * cout);
      | }
      ClassDeclTypeOptions=|
      | C[1 1]@t132@namespace DoubleStream {
      | template < int NSamples, int ShiftAcc, bool DiscardSample, bool SwapRead > class FIR_MultiKernel_cincout;
      | }
      ClassDecl=|
      | namespace DoubleStream {
      | template < int NSamples, int ShiftAcc, bool DiscardSample, bool SwapRead > class FIR_MultiKernel_cincout;
      | }
  filter37 : ModelComposer/AIE Class Kernel  KernelAllAttrs=|  PortNames={'sin1'; 'sin2'; 'cin'; 'cout'}  PortSerializedTypes={'{Q2{P{Tinput_stream{1{t{Scint16}}}}}}'; '{Q2{P{Tinput_stream{1{t{Scint16}}}}}}'; '{P{Tinput_stream{1{t{Scacc48_t}}}}}'; '{P{Toutput_stream{1{t{Scacc48_t}}}}}'}  PortWindowSizes={0.000000000000000000e+00; 0.000000000000000000e+00; 0.000000000000000000e+00; 0.000000000000000000e+00}  PortWindowMargins={0.000000000000000000e+00; 0.000000000000000000e+00; 0.000000000000000000e+00; 0.000000000000000000e+00}  PortSynchronicities={'auto'; 'auto'; 'auto'; 'auto'}  PortSignalSizes={0.000000000000000000e+00; 0.000000000000000000e+00; 0.000000000000000000e+00; 8.000000000000000000e+00}  ClassTemplateSpecKind=implicit  ClassTemplateParamNames={'NSamples'; 'ShiftAcc'; 'DiscardSample'; 'SwapRead'}  ClassTemplateParamKinds={'nontype'; 'nontype'; 'nontype'; 'nontype'}  ClassTemplateParamTypes={'int'; 'int'; 'bool'; 'bool'}  ClassTemplateParamValues={'512', '15', '0', '0'}  ClassCtorParamNames={'taps'}  ClassCtorParamSerializedTypes={'{R{Q1{C{Scint16}4}}}'}  ClassCtorParamValues={'[-54-21i 102-525i 8773-2748i 342+439i]'}  ClassIndex=1  ClassCtorIndex=1  ClassTabVisible=on  ClassTemplateParamsVisible=on  ClassCtorDeclVisible=on  ClassCtorParamsVisible=on  FunctionTabVisible=on  FunctionDecl=|  PortAttrs={ 'input', 'sin1', 'input_stream_cint16 * restrict', '', '', '', ''; 'input', 'sin2', 'input_stream_cint16 * restrict', '', '', '', ''; 'input', 'cin', 'input_stream< cacc48_t > *', '', '', '', ''; 'output', 'cout', 'output_stream< cacc48_t > *', '', '', '', 'OUTPUT_SIZE' }  PortAttrsEnables={'off', 'off', 'off', 'off', 'off', 'off', 'off';'off', 'off', 'off', 'off', 'off', 'off', 'off';'off', 'off', 'off', 'off', 'off', 'off', 'off';'off', 'off', 'off', 'off', 'off', 'off', 'on'}  SampleTime=-1  ClassDeclTypeOptions=|  ClassDecl=|  ClassTemplateParams={ 'NSamples', 'int', 'BURST_LENGTH'; 'ShiftAcc', 'int', 'SHIFT_ACC'; 'DiscardSample', 'bool', 'FALSE'; 'SwapRead', 'bool', 'FALSE' }  ClassTemplateParamsEnables={'off', 'off', 'on';'off', 'off', 'on';'off', 'off', 'on';'off', 'off', 'on'}  ClassCtorDeclTypeOptions=C[1 1]@t54@FIR_MultiKernel_cincout(cint16 const ( & taps ) [ 4 ])  ClassCtorDecl=FIR_MultiKernel_cincout(cint16 const ( & taps ) [ 4 ])  ClassCtorParams={ 'taps', 'cint16 const ( &) [ 4 ]', 'phi_0' }  KernelHeaderFile=FirDoubleStream.h  KernelClassName=DoubleStream::FIR_MultiKernel_cincout  KernelFunction=filter  KernelSourceFile=FirDoubleStream.cpp  KernelSearchPaths={'$SRC/aie_kernels'}  PreProcOptions={}  CoreRuntimeRatio=0.9  KernelLocSpec=off  ColRowLocation=[0 0]  blockJsonConstraints="{\"type\":\"constraint\",\"constraintType\":\"coreUtilization\",\"sid\":\"57\",\"lhs\":{\"type\":\"runtimeRatio\",\"args\":{\"type\":\"kernel\",\"name\":\"DualStreamSSR_1/Subsystem/filter38\",\"sid\":\"57\"}},\"rhs\":{\"type\":\"evaluable\",\"expr\":\"0.9\",\"value\":0.9},\"equality\":true}"  deprecateConstraints=1
      KernelAllAttrs=|
      | s[12;12;9;9;19;14;21;23;24;21;12;24;26;26;26;27;28;9;21;23;23;23;24;25;14;19;19;29]@FunctionNameDeclFileNamePortNamesPortTypesPortSerializedTypesPortDirectionsPortWindowSizeEnablesPortWindowMarginEnablesPortSynchronicityEnablesPortSignalSizeEnablesFunctionDeclFunctionTemplateSpecKindFunctionTemplateParamNamesFunctionTemplateParamKindsFunctionTemplateParamTypesFunctionTemplateParamValuesFunctionTemplateParamEnablesClassDeclClassTemplateSpecKindClassTemplateParamNamesClassTemplateParamKindsClassTemplateParamTypesClassTemplateParamValuesClassTemplateParamEnablesClassCtorDeclsClassCtorParamNamesClassCtorParamTypesClassCtorParamSerializedTypes[1 1]@C[28 1]@t6@filtert42@../../../aie/aie_kernels/FirDoubleStream.hC[4 1]@t4@sin1t4@sin2t3@cint4@coutC[4 1]@t30@input_stream_cint16 * restrictt30@input_stream_cint16 * restrictt26@input_stream< cacc48_t > *t27@output_stream< cacc48_t > *C[4 1]@t37@{Q2{P{Tinput_stream{1{t{Scint16}}}}}}t37@{Q2{P{Tinput_stream{1{t{Scint16}}}}}}t35@{P{Tinput_stream{1{t{Scacc48_t}}}}}t36@{P{Toutput_stream{1{t{Scacc48_t}}}}}C[4 1]@t5@inputt5@inputt5@inputt6@outputC[4 1]@l0@l0@l0@l0@C[4 1]@l0@l0@l0@l0@C[4 1]@l0@l0@l0@l0@C[4 1]@l0@l0@l0@l1@t281@namespace DoubleStream {
      | template < int NSamples, int ShiftAcc, bool DiscardSample, bool SwapRead > 
      | void FIR_MultiKernel_cincout::
      | filter(input_stream_cint16 * restrict sin1, input_stream_cint16 * restrict sin2, input_stream< cacc48_t > * cin, output_stream< cacc48_t > * cout);
      | }t4@nonee[0 1]@e[0 1]@e[0 1]@e[0 1]@e[0 1]@t132@namespace DoubleStream {
      | template < int NSamples, int ShiftAcc, bool DiscardSample, bool SwapRead > class FIR_MultiKernel_cincout;
      | }t8@implicitC[4 1]@t8@NSamplest8@ShiftAcct13@DiscardSamplet8@SwapReadC[4 1]@t7@nontypet7@nontypet7@nontypet7@nontypeC[4 1]@t3@intt3@intt4@boolt4@boolC[4 1]@nnnnC[4 1]@l1@l1@l1@l1@C[1 1]@t54@FIR_MultiKernel_cincout(cint16 const ( & taps ) [ 4 ])C[1 1]@C[1 1]@t4@tapsC[1 1]@C[1 1]@t23@cint16 const ( &) [ 4 ]C[1 1]@C[1 1]@t20@{R{Q1{C{Scint16}4}}}
      FunctionDecl=|
      | namespace DoubleStream {
      | template < int NSamples, int ShiftAcc, bool DiscardSample, bool SwapRead > 
      | void FIR_MultiKernel_cincout::
      | filter(input_stream_cint16 * restrict sin1, input_stream_cint16 * restrict sin2, input_stream< cacc48_t > * cin, output_stream< cacc48_t > * cout);
      | }
      ClassDeclTypeOptions=|
      | C[1 1]@t132@namespace DoubleStream {
      | template < int NSamples, int ShiftAcc, bool DiscardSample, bool SwapRead > class FIR_MultiKernel_cincout;
      | }
      ClassDecl=|
      | namespace DoubleStream {
      | template < int NSamples, int ShiftAcc, bool DiscardSample, bool SwapRead > class FIR_MultiKernel_cincout;
      | }
  filter38 : ModelComposer/AIE Class Kernel  KernelAllAttrs=|  PortNames={'sin1'; 'sin2'; 'cin'; 'cout'}  PortSerializedTypes={'{Q2{P{Tinput_stream{1{t{Scint16}}}}}}'; '{Q2{P{Tinput_stream{1{t{Scint16}}}}}}'; '{P{Tinput_stream{1{t{Scacc48_t}}}}}'; '{P{Toutput_stream{1{t{Scacc48_t}}}}}'}  PortWindowSizes={0.000000000000000000e+00; 0.000000000000000000e+00; 0.000000000000000000e+00; 0.000000000000000000e+00}  PortWindowMargins={0.000000000000000000e+00; 0.000000000000000000e+00; 0.000000000000000000e+00; 0.000000000000000000e+00}  PortSynchronicities={'auto'; 'auto'; 'auto'; 'auto'}  PortSignalSizes={0.000000000000000000e+00; 0.000000000000000000e+00; 0.000000000000000000e+00; 8.000000000000000000e+00}  ClassTemplateSpecKind=implicit  ClassTemplateParamNames={'NSamples'; 'ShiftAcc'; 'DiscardSample'; 'SwapRead'}  ClassTemplateParamKinds={'nontype'; 'nontype'; 'nontype'; 'nontype'}  ClassTemplateParamTypes={'int'; 'int'; 'bool'; 'bool'}  ClassTemplateParamValues={'512', '15', '1', '0'}  ClassCtorParamNames={'taps'}  ClassCtorParamSerializedTypes={'{R{Q1{C{Scint16}4}}}'}  ClassCtorParamValues={'[-121-233i 237-96i 1454+497i 14+121i]'}  ClassIndex=1  ClassCtorIndex=1  ClassTabVisible=on  ClassTemplateParamsVisible=on  ClassCtorDeclVisible=on  ClassCtorParamsVisible=on  FunctionTabVisible=on  FunctionDecl=|  PortAttrs={ 'input', 'sin1', 'input_stream_cint16 * restrict', '', '', '', ''; 'input', 'sin2', 'input_stream_cint16 * restrict', '', '', '', ''; 'input', 'cin', 'input_stream< cacc48_t > *', '', '', '', ''; 'output', 'cout', 'output_stream< cacc48_t > *', '', '', '', 'OUTPUT_SIZE' }  PortAttrsEnables={'off', 'off', 'off', 'off', 'off', 'off', 'off';'off', 'off', 'off', 'off', 'off', 'off', 'off';'off', 'off', 'off', 'off', 'off', 'off', 'off';'off', 'off', 'off', 'off', 'off', 'off', 'on'}  SampleTime=-1  ClassDeclTypeOptions=|  ClassDecl=|  ClassTemplateParams={ 'NSamples', 'int', 'BURST_LENGTH'; 'ShiftAcc', 'int', 'SHIFT_ACC'; 'DiscardSample', 'bool', 'TRUE'; 'SwapRead', 'bool', 'FALSE' }  ClassTemplateParamsEnables={'off', 'off', 'on';'off', 'off', 'on';'off', 'off', 'on';'off', 'off', 'on'}  ClassCtorDeclTypeOptions=C[1 1]@t54@FIR_MultiKernel_cincout(cint16 const ( & taps ) [ 4 ])  ClassCtorDecl=FIR_MultiKernel_cincout(cint16 const ( & taps ) [ 4 ])  ClassCtorParams={ 'taps', 'cint16 const ( &) [ 4 ]', 'phi_4' }  KernelHeaderFile=FirDoubleStream.h  KernelClassName=DoubleStream::FIR_MultiKernel_cincout  KernelFunction=filter  KernelSourceFile=FirDoubleStream.cpp  KernelSearchPaths={'$SRC/aie_kernels'}  PreProcOptions={}  CoreRuntimeRatio=0.9  KernelLocSpec=off  ColRowLocation=[0 0]  blockJsonConstraints="{\"type\":\"constraint\",\"constraintType\":\"coreUtilization\",\"sid\":\"57\",\"lhs\":{\"type\":\"runtimeRatio\",\"args\":{\"type\":\"kernel\",\"name\":\"DualStreamSSR_1/Subsystem/filter38\",\"sid\":\"57\"}},\"rhs\":{\"type\":\"evaluable\",\"expr\":\"0.9\",\"value\":0.9},\"equality\":true}"  deprecateConstraints=1
      KernelAllAttrs=|
      | s[12;12;9;9;19;14;21;23;24;21;12;24;26;26;26;27;28;9;21;23;23;23;24;25;14;19;19;29]@FunctionNameDeclFileNamePortNamesPortTypesPortSerializedTypesPortDirectionsPortWindowSizeEnablesPortWindowMarginEnablesPortSynchronicityEnablesPortSignalSizeEnablesFunctionDeclFunctionTemplateSpecKindFunctionTemplateParamNamesFunctionTemplateParamKindsFunctionTemplateParamTypesFunctionTemplateParamValuesFunctionTemplateParamEnablesClassDeclClassTemplateSpecKindClassTemplateParamNamesClassTemplateParamKindsClassTemplateParamTypesClassTemplateParamValuesClassTemplateParamEnablesClassCtorDeclsClassCtorParamNamesClassCtorParamTypesClassCtorParamSerializedTypes[1 1]@C[28 1]@t6@filtert42@../../../aie/aie_kernels/FirDoubleStream.hC[4 1]@t4@sin1t4@sin2t3@cint4@coutC[4 1]@t30@input_stream_cint16 * restrictt30@input_stream_cint16 * restrictt26@input_stream< cacc48_t > *t27@output_stream< cacc48_t > *C[4 1]@t37@{Q2{P{Tinput_stream{1{t{Scint16}}}}}}t37@{Q2{P{Tinput_stream{1{t{Scint16}}}}}}t35@{P{Tinput_stream{1{t{Scacc48_t}}}}}t36@{P{Toutput_stream{1{t{Scacc48_t}}}}}C[4 1]@t5@inputt5@inputt5@inputt6@outputC[4 1]@l0@l0@l0@l0@C[4 1]@l0@l0@l0@l0@C[4 1]@l0@l0@l0@l0@C[4 1]@l0@l0@l0@l1@t281@namespace DoubleStream {
      | template < int NSamples, int ShiftAcc, bool DiscardSample, bool SwapRead > 
      | void FIR_MultiKernel_cincout::
      | filter(input_stream_cint16 * restrict sin1, input_stream_cint16 * restrict sin2, input_stream< cacc48_t > * cin, output_stream< cacc48_t > * cout);
      | }t4@nonee[0 1]@e[0 1]@e[0 1]@e[0 1]@e[0 1]@t132@namespace DoubleStream {
      | template < int NSamples, int ShiftAcc, bool DiscardSample, bool SwapRead > class FIR_MultiKernel_cincout;
      | }t8@implicitC[4 1]@t8@NSamplest8@ShiftAcct13@DiscardSamplet8@SwapReadC[4 1]@t7@nontypet7@nontypet7@nontypet7@nontypeC[4 1]@t3@intt3@intt4@boolt4@boolC[4 1]@nnnnC[4 1]@l1@l1@l1@l1@C[1 1]@t54@FIR_MultiKernel_cincout(cint16 const ( & taps ) [ 4 ])C[1 1]@C[1 1]@t4@tapsC[1 1]@C[1 1]@t23@cint16 const ( &) [ 4 ]C[1 1]@C[1 1]@t20@{R{Q1{C{Scint16}4}}}
      FunctionDecl=|
      | namespace DoubleStream {
      | template < int NSamples, int ShiftAcc, bool DiscardSample, bool SwapRead > 
      | void FIR_MultiKernel_cincout::
      | filter(input_stream_cint16 * restrict sin1, input_stream_cint16 * restrict sin2, input_stream< cacc48_t > * cin, output_stream< cacc48_t > * cout);
      | }
      ClassDeclTypeOptions=|
      | C[1 1]@t132@namespace DoubleStream {
      | template < int NSamples, int ShiftAcc, bool DiscardSample, bool SwapRead > class FIR_MultiKernel_cincout;
      | }
      ClassDecl=|
      | namespace DoubleStream {
      | template < int NSamples, int ShiftAcc, bool DiscardSample, bool SwapRead > class FIR_MultiKernel_cincout;
      | }
  filter39 : ModelComposer/AIE Class Kernel  KernelAllAttrs=|  PortNames={'sin1'; 'sin2'; 'cin'; 'sout1'; 'sout2'}  PortSerializedTypes={'{Q2{P{Tinput_stream{1{t{Scint16}}}}}}'; '{Q2{P{Tinput_stream{1{t{Scint16}}}}}}'; '{P{Tinput_stream{1{t{Scacc48_t}}}}}'; '{Q2{P{Toutput_stream{1{t{Scint16}}}}}}'; '{Q2{P{Toutput_stream{1{t{Scint16}}}}}}'}  PortWindowSizes={0.000000000000000000e+00; 0.000000000000000000e+00; 0.000000000000000000e+00; 0.000000000000000000e+00; 0.000000000000000000e+00}  PortWindowMargins={0.000000000000000000e+00; 0.000000000000000000e+00; 0.000000000000000000e+00; 0.000000000000000000e+00; 0.000000000000000000e+00}  PortSynchronicities={'auto'; 'auto'; 'auto'; 'auto'; 'auto'}  PortSignalSizes={0.000000000000000000e+00; 0.000000000000000000e+00; 0.000000000000000000e+00; 4.000000000000000000e+00; 4.000000000000000000e+00}  ClassTemplateSpecKind=implicit  ClassTemplateParamNames={'NSamples'; 'ShiftAcc'; 'DiscardSample'; 'SwapRead'}  ClassTemplateParamKinds={'nontype'; 'nontype'; 'nontype'; 'nontype'}  ClassTemplateParamTypes={'int'; 'int'; 'bool'; 'bool'}  ClassTemplateParamValues={'512', '15', '1', '0'}  ClassCtorParamNames={'taps'}  ClassCtorParamSerializedTypes={'{R{Q1{C{Scint16}4}}}'}  ClassCtorParamValues={'[14-121i 1454-497i 237+96i -121+233i]'}  ClassIndex=1  ClassCtorIndex=1  ClassTabVisible=on  ClassTemplateParamsVisible=on  ClassCtorDeclVisible=on  ClassCtorParamsVisible=on  FunctionTabVisible=on  FunctionDecl=|  PortAttrs={ 'input', 'sin1', 'input_stream_cint16 * restrict', '', '', '', ''; 'input', 'sin2', 'input_stream_cint16 * restrict', '', '', '', ''; 'input', 'cin', 'input_stream< cacc48_t > *', '', '', '', ''; 'output', 'sout1', 'output_stream_cint16 * restrict', '', '', '', 'OUTPUT_SIZE/2'; 'output', 'sout2', 'output_stream_cint16 * restrict', '', '', '', 'OUTPUT_SIZE/2' }  PortAttrsEnables={'off', 'off', 'off', 'off', 'off', 'off', 'off';'off', 'off', 'off', 'off', 'off', 'off', 'off';'off', 'off', 'off', 'off', 'off', 'off', 'off';'off', 'off', 'off', 'off', 'off', 'off', 'on';'off', 'off', 'off', 'off', 'off', 'off', 'on'}  SampleTime=-1  ClassDeclTypeOptions=|  ClassDecl=|  ClassTemplateParams={ 'NSamples', 'int', 'BURST_LENGTH'; 'ShiftAcc', 'int', 'SHIFT_ACC'; 'DiscardSample', 'bool', 'TRUE'; 'SwapRead', 'bool', 'FALSE' }  ClassTemplateParamsEnables={'off', 'off', 'on';'off', 'off', 'on';'off', 'off', 'on';'off', 'off', 'on'}  ClassCtorDeclTypeOptions=C[1 1]@t50@FIR_MultiKernel_cin(cint16 const ( & taps ) [ 4 ])  ClassCtorDecl=FIR_MultiKernel_cin(cint16 const ( & taps ) [ 4 ])  ClassCtorParams={ 'taps', 'cint16 const ( &) [ 4 ]', 'phi_3' }  KernelHeaderFile=FirDoubleStream.h  KernelClassName=DoubleStream::FIR_MultiKernel_cin  KernelFunction=filter  KernelSourceFile=FirDoubleStream.cpp  KernelSearchPaths={'$SRC/aie_kernels'}  PreProcOptions={}  CoreRuntimeRatio=0.9  KernelLocSpec=off  ColRowLocation=[0 0]  blockJsonConstraints="{\"type\":\"constraint\",\"constraintType\":\"coreUtilization\",\"sid\":\"58\",\"lhs\":{\"type\":\"runtimeRatio\",\"args\":{\"type\":\"kernel\",\"name\":\"DualStreamSSR_1/Subsystem/filter39\",\"sid\":\"58\"}},\"rhs\":{\"type\":\"evaluable\",\"expr\":\"0.9\",\"value\":0.9},\"equality\":true}"  deprecateConstraints=1
      KernelAllAttrs=|
      | s[12;12;9;9;19;14;21;23;24;21;12;24;26;26;26;27;28;9;21;23;23;23;24;25;14;19;19;29]@FunctionNameDeclFileNamePortNamesPortTypesPortSerializedTypesPortDirectionsPortWindowSizeEnablesPortWindowMarginEnablesPortSynchronicityEnablesPortSignalSizeEnablesFunctionDeclFunctionTemplateSpecKindFunctionTemplateParamNamesFunctionTemplateParamKindsFunctionTemplateParamTypesFunctionTemplateParamValuesFunctionTemplateParamEnablesClassDeclClassTemplateSpecKindClassTemplateParamNamesClassTemplateParamKindsClassTemplateParamTypesClassTemplateParamValuesClassTemplateParamEnablesClassCtorDeclsClassCtorParamNamesClassCtorParamTypesClassCtorParamSerializedTypes[1 1]@C[28 1]@t6@filtert42@../../../aie/aie_kernels/FirDoubleStream.hC[5 1]@t4@sin1t4@sin2t3@cint5@sout1t5@sout2C[5 1]@t30@input_stream_cint16 * restrictt30@input_stream_cint16 * restrictt26@input_stream< cacc48_t > *t31@output_stream_cint16 * restrictt31@output_stream_cint16 * restrictC[5 1]@t37@{Q2{P{Tinput_stream{1{t{Scint16}}}}}}t37@{Q2{P{Tinput_stream{1{t{Scint16}}}}}}t35@{P{Tinput_stream{1{t{Scacc48_t}}}}}t38@{Q2{P{Toutput_stream{1{t{Scint16}}}}}}t38@{Q2{P{Toutput_stream{1{t{Scint16}}}}}}C[5 1]@t5@inputt5@inputt5@inputt6@outputt6@outputC[5 1]@l0@l0@l0@l0@l0@C[5 1]@l0@l0@l0@l0@l0@C[5 1]@l0@l0@l0@l0@l0@C[5 1]@l0@l0@l0@l1@l1@t321@namespace DoubleStream {
      | template < int NSamples, int ShiftAcc, bool DiscardSample, bool SwapRead > 
      | void FIR_MultiKernel_cin::
      | filter(input_stream_cint16 * restrict sin1, input_stream_cint16 * restrict sin2, input_stream< cacc48_t > * cin, output_stream_cint16 * restrict sout1, output_stream_cint16 * restrict sout2);
      | }t4@nonee[0 1]@e[0 1]@e[0 1]@e[0 1]@e[0 1]@t128@namespace DoubleStream {
      | template < int NSamples, int ShiftAcc, bool DiscardSample, bool SwapRead > class FIR_MultiKernel_cin;
      | }t8@implicitC[4 1]@t8@NSamplest8@ShiftAcct13@DiscardSamplet8@SwapReadC[4 1]@t7@nontypet7@nontypet7@nontypet7@nontypeC[4 1]@t3@intt3@intt4@boolt4@boolC[4 1]@nnnnC[4 1]@l1@l1@l1@l1@C[1 1]@t50@FIR_MultiKernel_cin(cint16 const ( & taps ) [ 4 ])C[1 1]@C[1 1]@t4@tapsC[1 1]@C[1 1]@t23@cint16 const ( &) [ 4 ]C[1 1]@C[1 1]@t20@{R{Q1{C{Scint16}4}}}
      FunctionDecl=|
      | namespace DoubleStream {
      | template < int NSamples, int ShiftAcc, bool DiscardSample, bool SwapRead > 
      | void FIR_MultiKernel_cin::
      | filter(input_stream_cint16 * restrict sin1, input_stream_cint16 * restrict sin2, input_stream< cacc48_t > * cin, output_stream_cint16 * restrict sout1, output_stream_cint16 * restrict sout2);
      | }
      ClassDeclTypeOptions=|
      | C[1 1]@t128@namespace DoubleStream {
      | template < int NSamples, int ShiftAcc, bool DiscardSample, bool SwapRead > class FIR_MultiKernel_cin;
      | }
      ClassDecl=|
      | namespace DoubleStream {
      | template < int NSamples, int ShiftAcc, bool DiscardSample, bool SwapRead > class FIR_MultiKernel_cin;
      | }
  filter4 : ModelComposer/AIE Class Kernel  KernelAllAttrs=|  PortNames={'sin1'; 'sin2'; 'cin'; 'cout'}  PortSerializedTypes={'{Q2{P{Tinput_stream{1{t{Scint16}}}}}}'; '{Q2{P{Tinput_stream{1{t{Scint16}}}}}}'; '{P{Tinput_stream{1{t{Scacc48_t}}}}}'; '{P{Toutput_stream{1{t{Scacc48_t}}}}}'}  PortWindowSizes={0.000000000000000000e+00; 0.000000000000000000e+00; 0.000000000000000000e+00; 0.000000000000000000e+00}  PortWindowMargins={0.000000000000000000e+00; 0.000000000000000000e+00; 0.000000000000000000e+00; 0.000000000000000000e+00}  PortSynchronicities={'auto'; 'auto'; 'auto'; 'auto'}  PortSignalSizes={0.000000000000000000e+00; 0.000000000000000000e+00; 0.000000000000000000e+00; 8.000000000000000000e+00}  ClassTemplateSpecKind=implicit  ClassTemplateParamNames={'NSamples'; 'ShiftAcc'; 'DiscardSample'; 'SwapRead'}  ClassTemplateParamKinds={'nontype'; 'nontype'; 'nontype'; 'nontype'}  ClassTemplateParamTypes={'int'; 'int'; 'bool'; 'bool'}  ClassTemplateParamValues={'512', '15', '0', '0'}  ClassCtorParamNames={'taps'}  ClassCtorParamSerializedTypes={'{R{Q1{C{Scint16}4}}}'}  ClassCtorParamValues={'[-121-233i 237-96i 1454+497i 14+121i]'}  ClassIndex=1  ClassCtorIndex=1  ClassTabVisible=on  ClassTemplateParamsVisible=on  ClassCtorDeclVisible=on  ClassCtorParamsVisible=on  FunctionTabVisible=on  FunctionDecl=|  PortAttrs={ 'input', 'sin1', 'input_stream_cint16 * restrict', '', '', '', ''; 'input', 'sin2', 'input_stream_cint16 * restrict', '', '', '', ''; 'input', 'cin', 'input_stream< cacc48_t > *', '', '', '', ''; 'output', 'cout', 'output_stream< cacc48_t > *', '', '', '', 'OUTPUT_SIZE' }  PortAttrsEnables={'off', 'off', 'off', 'off', 'off', 'off', 'off';'off', 'off', 'off', 'off', 'off', 'off', 'off';'off', 'off', 'off', 'off', 'off', 'off', 'off';'off', 'off', 'off', 'off', 'off', 'off', 'on'}  SampleTime=-1  ClassDeclTypeOptions=|  ClassDecl=|  ClassTemplateParams={ 'NSamples', 'int', 'BURST_LENGTH'; 'ShiftAcc', 'int', 'SHIFT_ACC'; 'DiscardSample', 'bool', 'FALSE'; 'SwapRead', 'bool', 'FALSE' }  ClassTemplateParamsEnables={'off', 'off', 'on';'off', 'off', 'on';'off', 'off', 'on';'off', 'off', 'on'}  ClassCtorDeclTypeOptions=C[1 1]@t54@FIR_MultiKernel_cincout(cint16 const ( & taps ) [ 4 ])  ClassCtorDecl=FIR_MultiKernel_cincout(cint16 const ( & taps ) [ 4 ])  ClassCtorParams={ 'taps', 'cint16 const ( &) [ 4 ]', 'phi_4' }  KernelHeaderFile=FirDoubleStream.h  KernelClassName=DoubleStream::FIR_MultiKernel_cincout  KernelFunction=filter  KernelSourceFile=FirDoubleStream.cpp  KernelSearchPaths={'$SRC/aie_kernels'}  PreProcOptions={}  CoreRuntimeRatio=0.9  KernelLocSpec=off  ColRowLocation=[0 0]  blockJsonConstraints="{\"type\":\"constraint\",\"constraintType\":\"coreUtilization\",\"sid\":\"2\",\"lhs\":{\"type\":\"runtimeRatio\",\"args\":{\"type\":\"kernel\",\"name\":\"DualStreamSSR_1/Subsystem/filter1\",\"sid\":\"2\"}},\"rhs\":{\"type\":\"evaluable\",\"expr\":\"0.9\",\"value\":0.9},\"equality\":true}"  deprecateConstraints=1
      KernelAllAttrs=|
      | s[12;12;9;9;19;14;21;23;24;21;12;24;26;26;26;27;28;9;21;23;23;23;24;25;14;19;19;29]@FunctionNameDeclFileNamePortNamesPortTypesPortSerializedTypesPortDirectionsPortWindowSizeEnablesPortWindowMarginEnablesPortSynchronicityEnablesPortSignalSizeEnablesFunctionDeclFunctionTemplateSpecKindFunctionTemplateParamNamesFunctionTemplateParamKindsFunctionTemplateParamTypesFunctionTemplateParamValuesFunctionTemplateParamEnablesClassDeclClassTemplateSpecKindClassTemplateParamNamesClassTemplateParamKindsClassTemplateParamTypesClassTemplateParamValuesClassTemplateParamEnablesClassCtorDeclsClassCtorParamNamesClassCtorParamTypesClassCtorParamSerializedTypes[1 1]@C[28 1]@t6@filtert42@../../../aie/aie_kernels/FirDoubleStream.hC[4 1]@t4@sin1t4@sin2t3@cint4@coutC[4 1]@t30@input_stream_cint16 * restrictt30@input_stream_cint16 * restrictt26@input_stream< cacc48_t > *t27@output_stream< cacc48_t > *C[4 1]@t37@{Q2{P{Tinput_stream{1{t{Scint16}}}}}}t37@{Q2{P{Tinput_stream{1{t{Scint16}}}}}}t35@{P{Tinput_stream{1{t{Scacc48_t}}}}}t36@{P{Toutput_stream{1{t{Scacc48_t}}}}}C[4 1]@t5@inputt5@inputt5@inputt6@outputC[4 1]@l0@l0@l0@l0@C[4 1]@l0@l0@l0@l0@C[4 1]@l0@l0@l0@l0@C[4 1]@l0@l0@l0@l1@t281@namespace DoubleStream {
      | template < int NSamples, int ShiftAcc, bool DiscardSample, bool SwapRead > 
      | void FIR_MultiKernel_cincout::
      | filter(input_stream_cint16 * restrict sin1, input_stream_cint16 * restrict sin2, input_stream< cacc48_t > * cin, output_stream< cacc48_t > * cout);
      | }t4@nonee[0 1]@e[0 1]@e[0 1]@e[0 1]@e[0 1]@t132@namespace DoubleStream {
      | template < int NSamples, int ShiftAcc, bool DiscardSample, bool SwapRead > class FIR_MultiKernel_cincout;
      | }t8@implicitC[4 1]@t8@NSamplest8@ShiftAcct13@DiscardSamplet8@SwapReadC[4 1]@t7@nontypet7@nontypet7@nontypet7@nontypeC[4 1]@t3@intt3@intt4@boolt4@boolC[4 1]@nnnnC[4 1]@l1@l1@l1@l1@C[1 1]@t54@FIR_MultiKernel_cincout(cint16 const ( & taps ) [ 4 ])C[1 1]@C[1 1]@t4@tapsC[1 1]@C[1 1]@t23@cint16 const ( &) [ 4 ]C[1 1]@C[1 1]@t20@{R{Q1{C{Scint16}4}}}
      FunctionDecl=|
      | namespace DoubleStream {
      | template < int NSamples, int ShiftAcc, bool DiscardSample, bool SwapRead > 
      | void FIR_MultiKernel_cincout::
      | filter(input_stream_cint16 * restrict sin1, input_stream_cint16 * restrict sin2, input_stream< cacc48_t > * cin, output_stream< cacc48_t > * cout);
      | }
      ClassDeclTypeOptions=|
      | C[1 1]@t132@namespace DoubleStream {
      | template < int NSamples, int ShiftAcc, bool DiscardSample, bool SwapRead > class FIR_MultiKernel_cincout;
      | }
      ClassDecl=|
      | namespace DoubleStream {
      | template < int NSamples, int ShiftAcc, bool DiscardSample, bool SwapRead > class FIR_MultiKernel_cincout;
      | }
  filter40 : ModelComposer/AIE Class Kernel  KernelAllAttrs=|  PortNames={'sin1'; 'sin2'; 'cout'}  PortSerializedTypes={'{Q2{P{Tinput_stream{1{t{Scint16}}}}}}'; '{Q2{P{Tinput_stream{1{t{Scint16}}}}}}'; '{P{Toutput_stream{1{t{Scacc48_t}}}}}'}  PortWindowSizes={0.000000000000000000e+00; 0.000000000000000000e+00; 0.000000000000000000e+00}  PortWindowMargins={0.000000000000000000e+00; 0.000000000000000000e+00; 0.000000000000000000e+00}  PortSynchronicities={'auto'; 'auto'; 'auto'}  PortSignalSizes={0.000000000000000000e+00; 0.000000000000000000e+00; 8.000000000000000000e+00}  ClassTemplateSpecKind=implicit  ClassTemplateParamNames={'NSamples'; 'ShiftAcc'; 'DiscardSample'; 'SwapRead'}  ClassTemplateParamKinds={'nontype'; 'nontype'; 'nontype'; 'nontype'}  ClassTemplateParamTypes={'int'; 'int'; 'bool'; 'bool'}  ClassTemplateParamValues={'512', '15', '1', '0'}  ClassCtorParamNames={'taps'}  ClassCtorParamSerializedTypes={'{R{Q1{C{Scint16}4}}}'}  ClassCtorParamValues={'[-21+26i 1183+239i 248-2878i -160+111i]'}  ClassIndex=1  ClassCtorIndex=1  ClassTabVisible=on  ClassTemplateParamsVisible=on  ClassCtorDeclVisible=on  ClassCtorParamsVisible=on  FunctionTabVisible=on  FunctionDecl=|  PortAttrs={ 'input', 'sin1', 'input_stream_cint16 * restrict', '', '', '', ''; 'input', 'sin2', 'input_stream_cint16 * restrict', '', '', '', ''; 'output', 'cout', 'output_stream< cacc48_t > *', '', '', '', 'OUTPUT_SIZE' }  PortAttrsEnables={'off', 'off', 'off', 'off', 'off', 'off', 'off';'off', 'off', 'off', 'off', 'off', 'off', 'off';'off', 'off', 'off', 'off', 'off', 'off', 'on'}  SampleTime=-1  ClassDeclTypeOptions=|  ClassDecl=|  ClassTemplateParams={ 'NSamples', 'int', 'BURST_LENGTH'; 'ShiftAcc', 'int', 'SHIFT_ACC'; 'DiscardSample', 'bool', 'TRUE'; 'SwapRead', 'bool', 'FALSE' }  ClassTemplateParamsEnables={'off', 'off', 'on';'off', 'off', 'on';'off', 'off', 'on';'off', 'off', 'on'}  ClassCtorDeclTypeOptions=C[1 1]@t51@FIR_MultiKernel_cout(cint16 const ( & taps ) [ 4 ])  ClassCtorDecl=FIR_MultiKernel_cout(cint16 const ( & taps ) [ 4 ])  ClassCtorParams={ 'taps', 'cint16 const ( &) [ 4 ]', 'phi_2' }  KernelHeaderFile=FirDoubleStream.h  KernelClassName=DoubleStream::FIR_MultiKernel_cout  KernelFunction=filter  KernelSourceFile=FirDoubleStream.cpp  KernelSearchPaths={'$SRC/aie_kernels'}  PreProcOptions={}  CoreRuntimeRatio=0.9  KernelLocSpec=off  ColRowLocation=[0 0]  blockJsonConstraints="[{\"type\":\"constraint\",\"constraintType\":\"coreUtilization\",\"sid\":\"59\",\"lhs\":{\"type\":\"runtimeRatio\",\"args\":{\"type\":\"kernel\",\"name\":\"DualStreamSSR_1/Subsystem/filter40\",\"sid\":\"59\"}},\"rhs\":{\"type\":\"evaluable\",\"expr\":\"0.9\",\"value\":0.9},\"equality\":true},{\"type\":\"constraint\",\"constraintType\":\"location_kernel\",\"sid\":\"59\",\"lhs\":{\"type\":\"location\",\"templParam\":\"kernel\",\"args\":{\"type\":\"kernel\",\"name\":\"DualStreamSSR_1/Subsystem/filter40\",\"sid\":\"59\"}},\"rhs\":{\"type\":\"tile\",\"args\":[{\"type\":\"evaluable\",\"expr\":\"23\",\"value\":23},{\"type\":\"evaluable\",\"expr\":\"6\",\"value\":6}]},\"equality\":true}]"  deprecateConstraints=1
      KernelAllAttrs=|
      | s[12;12;9;9;19;14;21;23;24;21;12;24;26;26;26;27;28;9;21;23;23;23;24;25;14;19;19;29]@FunctionNameDeclFileNamePortNamesPortTypesPortSerializedTypesPortDirectionsPortWindowSizeEnablesPortWindowMarginEnablesPortSynchronicityEnablesPortSignalSizeEnablesFunctionDeclFunctionTemplateSpecKindFunctionTemplateParamNamesFunctionTemplateParamKindsFunctionTemplateParamTypesFunctionTemplateParamValuesFunctionTemplateParamEnablesClassDeclClassTemplateSpecKindClassTemplateParamNamesClassTemplateParamKindsClassTemplateParamTypesClassTemplateParamValuesClassTemplateParamEnablesClassCtorDeclsClassCtorParamNamesClassCtorParamTypesClassCtorParamSerializedTypes[1 1]@C[28 1]@t6@filtert42@../../../aie/aie_kernels/FirDoubleStream.hC[3 1]@t4@sin1t4@sin2t4@coutC[3 1]@t30@input_stream_cint16 * restrictt30@input_stream_cint16 * restrictt27@output_stream< cacc48_t > *C[3 1]@t37@{Q2{P{Tinput_stream{1{t{Scint16}}}}}}t37@{Q2{P{Tinput_stream{1{t{Scint16}}}}}}t36@{P{Toutput_stream{1{t{Scacc48_t}}}}}C[3 1]@t5@inputt5@inputt6@outputC[3 1]@l0@l0@l0@C[3 1]@l0@l0@l0@C[3 1]@l0@l0@l0@C[3 1]@l0@l0@l1@t246@namespace DoubleStream {
      | template < int NSamples, int ShiftAcc, bool DiscardSample, bool SwapRead > 
      | void FIR_MultiKernel_cout::
      | filter(input_stream_cint16 * restrict sin1, input_stream_cint16 * restrict sin2, output_stream< cacc48_t > * cout);
      | }t4@nonee[0 1]@e[0 1]@e[0 1]@e[0 1]@e[0 1]@t129@namespace DoubleStream {
      | template < int NSamples, int ShiftAcc, bool DiscardSample, bool SwapRead > class FIR_MultiKernel_cout;
      | }t8@implicitC[4 1]@t8@NSamplest8@ShiftAcct13@DiscardSamplet8@SwapReadC[4 1]@t7@nontypet7@nontypet7@nontypet7@nontypeC[4 1]@t3@intt3@intt4@boolt4@boolC[4 1]@nnnnC[4 1]@l1@l1@l1@l1@C[1 1]@t51@FIR_MultiKernel_cout(cint16 const ( & taps ) [ 4 ])C[1 1]@C[1 1]@t4@tapsC[1 1]@C[1 1]@t23@cint16 const ( &) [ 4 ]C[1 1]@C[1 1]@t20@{R{Q1{C{Scint16}4}}}
      FunctionDecl=|
      | namespace DoubleStream {
      | template < int NSamples, int ShiftAcc, bool DiscardSample, bool SwapRead > 
      | void FIR_MultiKernel_cout::
      | filter(input_stream_cint16 * restrict sin1, input_stream_cint16 * restrict sin2, output_stream< cacc48_t > * cout);
      | }
      ClassDeclTypeOptions=|
      | C[1 1]@t129@namespace DoubleStream {
      | template < int NSamples, int ShiftAcc, bool DiscardSample, bool SwapRead > class FIR_MultiKernel_cout;
      | }
      ClassDecl=|
      | namespace DoubleStream {
      | template < int NSamples, int ShiftAcc, bool DiscardSample, bool SwapRead > class FIR_MultiKernel_cout;
      | }
  filter41 : ModelComposer/AIE Class Kernel  KernelAllAttrs=|  PortNames={'sin1'; 'sin2'; 'cin'; 'cout'}  PortSerializedTypes={'{Q2{P{Tinput_stream{1{t{Scint16}}}}}}'; '{Q2{P{Tinput_stream{1{t{Scint16}}}}}}'; '{P{Tinput_stream{1{t{Scacc48_t}}}}}'; '{P{Toutput_stream{1{t{Scacc48_t}}}}}'}  PortWindowSizes={0.000000000000000000e+00; 0.000000000000000000e+00; 0.000000000000000000e+00; 0.000000000000000000e+00}  PortWindowMargins={0.000000000000000000e+00; 0.000000000000000000e+00; 0.000000000000000000e+00; 0.000000000000000000e+00}  PortSynchronicities={'auto'; 'auto'; 'auto'; 'auto'}  PortSignalSizes={0.000000000000000000e+00; 0.000000000000000000e+00; 0.000000000000000000e+00; 8.000000000000000000e+00}  ClassTemplateSpecKind=implicit  ClassTemplateParamNames={'NSamples'; 'ShiftAcc'; 'DiscardSample'; 'SwapRead'}  ClassTemplateParamKinds={'nontype'; 'nontype'; 'nontype'; 'nontype'}  ClassTemplateParamTypes={'int'; 'int'; 'bool'; 'bool'}  ClassTemplateParamValues={'512', '15', '1', '0'}  ClassCtorParamNames={'taps'}  ClassCtorParamSerializedTypes={'{R{Q1{C{Scint16}4}}}'}  ClassCtorParamValues={'[14-121i 1454-497i 237+96i -121+233i]'}  ClassIndex=1  ClassCtorIndex=1  ClassTabVisible=on  ClassTemplateParamsVisible=on  ClassCtorDeclVisible=on  ClassCtorParamsVisible=on  FunctionTabVisible=on  FunctionDecl=|  PortAttrs={ 'input', 'sin1', 'input_stream_cint16 * restrict', '', '', '', ''; 'input', 'sin2', 'input_stream_cint16 * restrict', '', '', '', ''; 'input', 'cin', 'input_stream< cacc48_t > *', '', '', '', ''; 'output', 'cout', 'output_stream< cacc48_t > *', '', '', '', 'OUTPUT_SIZE' }  PortAttrsEnables={'off', 'off', 'off', 'off', 'off', 'off', 'off';'off', 'off', 'off', 'off', 'off', 'off', 'off';'off', 'off', 'off', 'off', 'off', 'off', 'off';'off', 'off', 'off', 'off', 'off', 'off', 'on'}  SampleTime=-1  ClassDeclTypeOptions=|  ClassDecl=|  ClassTemplateParams={ 'NSamples', 'int', 'BURST_LENGTH'; 'ShiftAcc', 'int', 'SHIFT_ACC'; 'DiscardSample', 'bool', 'TRUE'; 'SwapRead', 'bool', 'FALSE' }  ClassTemplateParamsEnables={'off', 'off', 'on';'off', 'off', 'on';'off', 'off', 'on';'off', 'off', 'on'}  ClassCtorDeclTypeOptions=C[1 1]@t54@FIR_MultiKernel_cincout(cint16 const ( & taps ) [ 4 ])  ClassCtorDecl=FIR_MultiKernel_cincout(cint16 const ( & taps ) [ 4 ])  ClassCtorParams={ 'taps', 'cint16 const ( &) [ 4 ]', 'phi_3' }  KernelHeaderFile=FirDoubleStream.h  KernelClassName=DoubleStream::FIR_MultiKernel_cincout  KernelFunction=filter  KernelSourceFile=FirDoubleStream.cpp  KernelSearchPaths={'$SRC/aie_kernels'}  PreProcOptions={}  CoreRuntimeRatio=0.9  KernelLocSpec=off  ColRowLocation=[0 0]  blockJsonConstraints="{\"type\":\"constraint\",\"constraintType\":\"coreUtilization\",\"sid\":\"60\",\"lhs\":{\"type\":\"runtimeRatio\",\"args\":{\"type\":\"kernel\",\"name\":\"DualStreamSSR_1/Subsystem/filter41\",\"sid\":\"60\"}},\"rhs\":{\"type\":\"evaluable\",\"expr\":\"0.9\",\"value\":0.9},\"equality\":true}"  deprecateConstraints=1
      KernelAllAttrs=|
      | s[12;12;9;9;19;14;21;23;24;21;12;24;26;26;26;27;28;9;21;23;23;23;24;25;14;19;19;29]@FunctionNameDeclFileNamePortNamesPortTypesPortSerializedTypesPortDirectionsPortWindowSizeEnablesPortWindowMarginEnablesPortSynchronicityEnablesPortSignalSizeEnablesFunctionDeclFunctionTemplateSpecKindFunctionTemplateParamNamesFunctionTemplateParamKindsFunctionTemplateParamTypesFunctionTemplateParamValuesFunctionTemplateParamEnablesClassDeclClassTemplateSpecKindClassTemplateParamNamesClassTemplateParamKindsClassTemplateParamTypesClassTemplateParamValuesClassTemplateParamEnablesClassCtorDeclsClassCtorParamNamesClassCtorParamTypesClassCtorParamSerializedTypes[1 1]@C[28 1]@t6@filtert42@../../../aie/aie_kernels/FirDoubleStream.hC[4 1]@t4@sin1t4@sin2t3@cint4@coutC[4 1]@t30@input_stream_cint16 * restrictt30@input_stream_cint16 * restrictt26@input_stream< cacc48_t > *t27@output_stream< cacc48_t > *C[4 1]@t37@{Q2{P{Tinput_stream{1{t{Scint16}}}}}}t37@{Q2{P{Tinput_stream{1{t{Scint16}}}}}}t35@{P{Tinput_stream{1{t{Scacc48_t}}}}}t36@{P{Toutput_stream{1{t{Scacc48_t}}}}}C[4 1]@t5@inputt5@inputt5@inputt6@outputC[4 1]@l0@l0@l0@l0@C[4 1]@l0@l0@l0@l0@C[4 1]@l0@l0@l0@l0@C[4 1]@l0@l0@l0@l1@t281@namespace DoubleStream {
      | template < int NSamples, int ShiftAcc, bool DiscardSample, bool SwapRead > 
      | void FIR_MultiKernel_cincout::
      | filter(input_stream_cint16 * restrict sin1, input_stream_cint16 * restrict sin2, input_stream< cacc48_t > * cin, output_stream< cacc48_t > * cout);
      | }t4@nonee[0 1]@e[0 1]@e[0 1]@e[0 1]@e[0 1]@t132@namespace DoubleStream {
      | template < int NSamples, int ShiftAcc, bool DiscardSample, bool SwapRead > class FIR_MultiKernel_cincout;
      | }t8@implicitC[4 1]@t8@NSamplest8@ShiftAcct13@DiscardSamplet8@SwapReadC[4 1]@t7@nontypet7@nontypet7@nontypet7@nontypeC[4 1]@t3@intt3@intt4@boolt4@boolC[4 1]@nnnnC[4 1]@l1@l1@l1@l1@C[1 1]@t54@FIR_MultiKernel_cincout(cint16 const ( & taps ) [ 4 ])C[1 1]@C[1 1]@t4@tapsC[1 1]@C[1 1]@t23@cint16 const ( &) [ 4 ]C[1 1]@C[1 1]@t20@{R{Q1{C{Scint16}4}}}
      FunctionDecl=|
      | namespace DoubleStream {
      | template < int NSamples, int ShiftAcc, bool DiscardSample, bool SwapRead > 
      | void FIR_MultiKernel_cincout::
      | filter(input_stream_cint16 * restrict sin1, input_stream_cint16 * restrict sin2, input_stream< cacc48_t > * cin, output_stream< cacc48_t > * cout);
      | }
      ClassDeclTypeOptions=|
      | C[1 1]@t132@namespace DoubleStream {
      | template < int NSamples, int ShiftAcc, bool DiscardSample, bool SwapRead > class FIR_MultiKernel_cincout;
      | }
      ClassDecl=|
      | namespace DoubleStream {
      | template < int NSamples, int ShiftAcc, bool DiscardSample, bool SwapRead > class FIR_MultiKernel_cincout;
      | }
  filter42 : ModelComposer/AIE Class Kernel  KernelAllAttrs=|  PortNames={'sin1'; 'sin2'; 'cin'; 'cout'}  PortSerializedTypes={'{Q2{P{Tinput_stream{1{t{Scint16}}}}}}'; '{Q2{P{Tinput_stream{1{t{Scint16}}}}}}'; '{P{Tinput_stream{1{t{Scacc48_t}}}}}'; '{P{Toutput_stream{1{t{Scacc48_t}}}}}'}  PortWindowSizes={0.000000000000000000e+00; 0.000000000000000000e+00; 0.000000000000000000e+00; 0.000000000000000000e+00}  PortWindowMargins={0.000000000000000000e+00; 0.000000000000000000e+00; 0.000000000000000000e+00; 0.000000000000000000e+00}  PortSynchronicities={'auto'; 'auto'; 'auto'; 'auto'}  PortSignalSizes={0.000000000000000000e+00; 0.000000000000000000e+00; 0.000000000000000000e+00; 8.000000000000000000e+00}  ClassTemplateSpecKind=implicit  ClassTemplateParamNames={'NSamples'; 'ShiftAcc'; 'DiscardSample'; 'SwapRead'}  ClassTemplateParamKinds={'nontype'; 'nontype'; 'nontype'; 'nontype'}  ClassTemplateParamTypes={'int'; 'int'; 'bool'; 'bool'}  ClassTemplateParamValues={'512', '15', '1', '0'}  ClassCtorParamNames={'taps'}  ClassCtorParamSerializedTypes={'{R{Q1{C{Scint16}4}}}'}  ClassCtorParamValues={'[-121-233i 237-96i 1454+497i 14+121i]'}  ClassIndex=1  ClassCtorIndex=1  ClassTabVisible=on  ClassTemplateParamsVisible=on  ClassCtorDeclVisible=on  ClassCtorParamsVisible=on  FunctionTabVisible=on  FunctionDecl=|  PortAttrs={ 'input', 'sin1', 'input_stream_cint16 * restrict', '', '', '', ''; 'input', 'sin2', 'input_stream_cint16 * restrict', '', '', '', ''; 'input', 'cin', 'input_stream< cacc48_t > *', '', '', '', ''; 'output', 'cout', 'output_stream< cacc48_t > *', '', '', '', 'OUTPUT_SIZE' }  PortAttrsEnables={'off', 'off', 'off', 'off', 'off', 'off', 'off';'off', 'off', 'off', 'off', 'off', 'off', 'off';'off', 'off', 'off', 'off', 'off', 'off', 'off';'off', 'off', 'off', 'off', 'off', 'off', 'on'}  SampleTime=-1  ClassDeclTypeOptions=|  ClassDecl=|  ClassTemplateParams={ 'NSamples', 'int', 'BURST_LENGTH'; 'ShiftAcc', 'int', 'SHIFT_ACC'; 'DiscardSample', 'bool', 'TRUE'; 'SwapRead', 'bool', 'FALSE' }  ClassTemplateParamsEnables={'off', 'off', 'on';'off', 'off', 'on';'off', 'off', 'on';'off', 'off', 'on'}  ClassCtorDeclTypeOptions=C[1 1]@t54@FIR_MultiKernel_cincout(cint16 const ( & taps ) [ 4 ])  ClassCtorDecl=FIR_MultiKernel_cincout(cint16 const ( & taps ) [ 4 ])  ClassCtorParams={ 'taps', 'cint16 const ( &) [ 4 ]', 'phi_4' }  KernelHeaderFile=FirDoubleStream.h  KernelClassName=DoubleStream::FIR_MultiKernel_cincout  KernelFunction=filter  KernelSourceFile=FirDoubleStream.cpp  KernelSearchPaths={'$SRC/aie_kernels'}  PreProcOptions={}  CoreRuntimeRatio=0.9  KernelLocSpec=off  ColRowLocation=[0 0]  blockJsonConstraints="{\"type\":\"constraint\",\"constraintType\":\"coreUtilization\",\"sid\":\"65\",\"lhs\":{\"type\":\"runtimeRatio\",\"args\":{\"type\":\"kernel\",\"name\":\"DualStreamSSR_1/Subsystem/filter46\",\"sid\":\"65\"}},\"rhs\":{\"type\":\"evaluable\",\"expr\":\"0.9\",\"value\":0.9},\"equality\":true}"  deprecateConstraints=1
      KernelAllAttrs=|
      | s[12;12;9;9;19;14;21;23;24;21;12;24;26;26;26;27;28;9;21;23;23;23;24;25;14;19;19;29]@FunctionNameDeclFileNamePortNamesPortTypesPortSerializedTypesPortDirectionsPortWindowSizeEnablesPortWindowMarginEnablesPortSynchronicityEnablesPortSignalSizeEnablesFunctionDeclFunctionTemplateSpecKindFunctionTemplateParamNamesFunctionTemplateParamKindsFunctionTemplateParamTypesFunctionTemplateParamValuesFunctionTemplateParamEnablesClassDeclClassTemplateSpecKindClassTemplateParamNamesClassTemplateParamKindsClassTemplateParamTypesClassTemplateParamValuesClassTemplateParamEnablesClassCtorDeclsClassCtorParamNamesClassCtorParamTypesClassCtorParamSerializedTypes[1 1]@C[28 1]@t6@filtert42@../../../aie/aie_kernels/FirDoubleStream.hC[4 1]@t4@sin1t4@sin2t3@cint4@coutC[4 1]@t30@input_stream_cint16 * restrictt30@input_stream_cint16 * restrictt26@input_stream< cacc48_t > *t27@output_stream< cacc48_t > *C[4 1]@t37@{Q2{P{Tinput_stream{1{t{Scint16}}}}}}t37@{Q2{P{Tinput_stream{1{t{Scint16}}}}}}t35@{P{Tinput_stream{1{t{Scacc48_t}}}}}t36@{P{Toutput_stream{1{t{Scacc48_t}}}}}C[4 1]@t5@inputt5@inputt5@inputt6@outputC[4 1]@l0@l0@l0@l0@C[4 1]@l0@l0@l0@l0@C[4 1]@l0@l0@l0@l0@C[4 1]@l0@l0@l0@l1@t281@namespace DoubleStream {
      | template < int NSamples, int ShiftAcc, bool DiscardSample, bool SwapRead > 
      | void FIR_MultiKernel_cincout::
      | filter(input_stream_cint16 * restrict sin1, input_stream_cint16 * restrict sin2, input_stream< cacc48_t > * cin, output_stream< cacc48_t > * cout);
      | }t4@nonee[0 1]@e[0 1]@e[0 1]@e[0 1]@e[0 1]@t132@namespace DoubleStream {
      | template < int NSamples, int ShiftAcc, bool DiscardSample, bool SwapRead > class FIR_MultiKernel_cincout;
      | }t8@implicitC[4 1]@t8@NSamplest8@ShiftAcct13@DiscardSamplet8@SwapReadC[4 1]@t7@nontypet7@nontypet7@nontypet7@nontypeC[4 1]@t3@intt3@intt4@boolt4@boolC[4 1]@nnnnC[4 1]@l1@l1@l1@l1@C[1 1]@t54@FIR_MultiKernel_cincout(cint16 const ( & taps ) [ 4 ])C[1 1]@C[1 1]@t4@tapsC[1 1]@C[1 1]@t23@cint16 const ( &) [ 4 ]C[1 1]@C[1 1]@t20@{R{Q1{C{Scint16}4}}}
      FunctionDecl=|
      | namespace DoubleStream {
      | template < int NSamples, int ShiftAcc, bool DiscardSample, bool SwapRead > 
      | void FIR_MultiKernel_cincout::
      | filter(input_stream_cint16 * restrict sin1, input_stream_cint16 * restrict sin2, input_stream< cacc48_t > * cin, output_stream< cacc48_t > * cout);
      | }
      ClassDeclTypeOptions=|
      | C[1 1]@t132@namespace DoubleStream {
      | template < int NSamples, int ShiftAcc, bool DiscardSample, bool SwapRead > class FIR_MultiKernel_cincout;
      | }
      ClassDecl=|
      | namespace DoubleStream {
      | template < int NSamples, int ShiftAcc, bool DiscardSample, bool SwapRead > class FIR_MultiKernel_cincout;
      | }
  filter43 : ModelComposer/AIE Class Kernel  KernelAllAttrs=|  PortNames={'sin1'; 'sin2'; 'cin'; 'cout'}  PortSerializedTypes={'{Q2{P{Tinput_stream{1{t{Scint16}}}}}}'; '{Q2{P{Tinput_stream{1{t{Scint16}}}}}}'; '{P{Tinput_stream{1{t{Scacc48_t}}}}}'; '{P{Toutput_stream{1{t{Scacc48_t}}}}}'}  PortWindowSizes={0.000000000000000000e+00; 0.000000000000000000e+00; 0.000000000000000000e+00; 0.000000000000000000e+00}  PortWindowMargins={0.000000000000000000e+00; 0.000000000000000000e+00; 0.000000000000000000e+00; 0.000000000000000000e+00}  PortSynchronicities={'auto'; 'auto'; 'auto'; 'auto'}  PortSignalSizes={0.000000000000000000e+00; 0.000000000000000000e+00; 0.000000000000000000e+00; 8.000000000000000000e+00}  ClassTemplateSpecKind=implicit  ClassTemplateParamNames={'NSamples'; 'ShiftAcc'; 'DiscardSample'; 'SwapRead'}  ClassTemplateParamKinds={'nontype'; 'nontype'; 'nontype'; 'nontype'}  ClassTemplateParamTypes={'int'; 'int'; 'bool'; 'bool'}  ClassTemplateParamValues={'512', '15', '1', '0'}  ClassCtorParamNames={'taps'}  ClassCtorParamSerializedTypes={'{R{Q1{C{Scint16}4}}}'}  ClassCtorParamValues={'[-160-111i 248+2878i 1183-239i -21-26i]'}  ClassIndex=1  ClassCtorIndex=1  ClassTabVisible=on  ClassTemplateParamsVisible=on  ClassCtorDeclVisible=on  ClassCtorParamsVisible=on  FunctionTabVisible=on  FunctionDecl=|  PortAttrs={ 'input', 'sin1', 'input_stream_cint16 * restrict', '', '', '', ''; 'input', 'sin2', 'input_stream_cint16 * restrict', '', '', '', ''; 'input', 'cin', 'input_stream< cacc48_t > *', '', '', '', ''; 'output', 'cout', 'output_stream< cacc48_t > *', '', '', '', 'OUTPUT_SIZE' }  PortAttrsEnables={'off', 'off', 'off', 'off', 'off', 'off', 'off';'off', 'off', 'off', 'off', 'off', 'off', 'off';'off', 'off', 'off', 'off', 'off', 'off', 'off';'off', 'off', 'off', 'off', 'off', 'off', 'on'}  SampleTime=-1  ClassDeclTypeOptions=|  ClassDecl=|  ClassTemplateParams={ 'NSamples', 'int', 'BURST_LENGTH'; 'ShiftAcc', 'int', 'SHIFT_ACC'; 'DiscardSample', 'bool', 'TRUE'; 'SwapRead', 'bool', 'FALSE' }  ClassTemplateParamsEnables={'off', 'off', 'on';'off', 'off', 'on';'off', 'off', 'on';'off', 'off', 'on'}  ClassCtorDeclTypeOptions=C[1 1]@t54@FIR_MultiKernel_cincout(cint16 const ( & taps ) [ 4 ])  ClassCtorDecl=FIR_MultiKernel_cincout(cint16 const ( & taps ) [ 4 ])  ClassCtorParams={ 'taps', 'cint16 const ( &) [ 4 ]', 'phi_5' }  KernelHeaderFile=FirDoubleStream.h  KernelClassName=DoubleStream::FIR_MultiKernel_cincout  KernelFunction=filter  KernelSourceFile=FirDoubleStream.cpp  KernelSearchPaths={'$SRC/aie_kernels'}  PreProcOptions={}  CoreRuntimeRatio=0.9  KernelLocSpec=off  ColRowLocation=[0 0]  blockJsonConstraints="{\"type\":\"constraint\",\"constraintType\":\"coreUtilization\",\"sid\":\"65\",\"lhs\":{\"type\":\"runtimeRatio\",\"args\":{\"type\":\"kernel\",\"name\":\"DualStreamSSR_1/Subsystem/filter46\",\"sid\":\"65\"}},\"rhs\":{\"type\":\"evaluable\",\"expr\":\"0.9\",\"value\":0.9},\"equality\":true}"  deprecateConstraints=1
      KernelAllAttrs=|
      | s[12;12;9;9;19;14;21;23;24;21;12;24;26;26;26;27;28;9;21;23;23;23;24;25;14;19;19;29]@FunctionNameDeclFileNamePortNamesPortTypesPortSerializedTypesPortDirectionsPortWindowSizeEnablesPortWindowMarginEnablesPortSynchronicityEnablesPortSignalSizeEnablesFunctionDeclFunctionTemplateSpecKindFunctionTemplateParamNamesFunctionTemplateParamKindsFunctionTemplateParamTypesFunctionTemplateParamValuesFunctionTemplateParamEnablesClassDeclClassTemplateSpecKindClassTemplateParamNamesClassTemplateParamKindsClassTemplateParamTypesClassTemplateParamValuesClassTemplateParamEnablesClassCtorDeclsClassCtorParamNamesClassCtorParamTypesClassCtorParamSerializedTypes[1 1]@C[28 1]@t6@filtert42@../../../aie/aie_kernels/FirDoubleStream.hC[4 1]@t4@sin1t4@sin2t3@cint4@coutC[4 1]@t30@input_stream_cint16 * restrictt30@input_stream_cint16 * restrictt26@input_stream< cacc48_t > *t27@output_stream< cacc48_t > *C[4 1]@t37@{Q2{P{Tinput_stream{1{t{Scint16}}}}}}t37@{Q2{P{Tinput_stream{1{t{Scint16}}}}}}t35@{P{Tinput_stream{1{t{Scacc48_t}}}}}t36@{P{Toutput_stream{1{t{Scacc48_t}}}}}C[4 1]@t5@inputt5@inputt5@inputt6@outputC[4 1]@l0@l0@l0@l0@C[4 1]@l0@l0@l0@l0@C[4 1]@l0@l0@l0@l0@C[4 1]@l0@l0@l0@l1@t281@namespace DoubleStream {
      | template < int NSamples, int ShiftAcc, bool DiscardSample, bool SwapRead > 
      | void FIR_MultiKernel_cincout::
      | filter(input_stream_cint16 * restrict sin1, input_stream_cint16 * restrict sin2, input_stream< cacc48_t > * cin, output_stream< cacc48_t > * cout);
      | }t4@nonee[0 1]@e[0 1]@e[0 1]@e[0 1]@e[0 1]@t132@namespace DoubleStream {
      | template < int NSamples, int ShiftAcc, bool DiscardSample, bool SwapRead > class FIR_MultiKernel_cincout;
      | }t8@implicitC[4 1]@t8@NSamplest8@ShiftAcct13@DiscardSamplet8@SwapReadC[4 1]@t7@nontypet7@nontypet7@nontypet7@nontypeC[4 1]@t3@intt3@intt4@boolt4@boolC[4 1]@nnnnC[4 1]@l1@l1@l1@l1@C[1 1]@t54@FIR_MultiKernel_cincout(cint16 const ( & taps ) [ 4 ])C[1 1]@C[1 1]@t4@tapsC[1 1]@C[1 1]@t23@cint16 const ( &) [ 4 ]C[1 1]@C[1 1]@t20@{R{Q1{C{Scint16}4}}}
      FunctionDecl=|
      | namespace DoubleStream {
      | template < int NSamples, int ShiftAcc, bool DiscardSample, bool SwapRead > 
      | void FIR_MultiKernel_cincout::
      | filter(input_stream_cint16 * restrict sin1, input_stream_cint16 * restrict sin2, input_stream< cacc48_t > * cin, output_stream< cacc48_t > * cout);
      | }
      ClassDeclTypeOptions=|
      | C[1 1]@t132@namespace DoubleStream {
      | template < int NSamples, int ShiftAcc, bool DiscardSample, bool SwapRead > class FIR_MultiKernel_cincout;
      | }
      ClassDecl=|
      | namespace DoubleStream {
      | template < int NSamples, int ShiftAcc, bool DiscardSample, bool SwapRead > class FIR_MultiKernel_cincout;
      | }
  filter44 : ModelComposer/AIE Class Kernel  KernelAllAttrs=|  PortNames={'sin1'; 'sin2'; 'cin'; 'cout'}  PortSerializedTypes={'{Q2{P{Tinput_stream{1{t{Scint16}}}}}}'; '{Q2{P{Tinput_stream{1{t{Scint16}}}}}}'; '{P{Tinput_stream{1{t{Scacc48_t}}}}}'; '{P{Toutput_stream{1{t{Scacc48_t}}}}}'}  PortWindowSizes={0.000000000000000000e+00; 0.000000000000000000e+00; 0.000000000000000000e+00; 0.000000000000000000e+00}  PortWindowMargins={0.000000000000000000e+00; 0.000000000000000000e+00; 0.000000000000000000e+00; 0.000000000000000000e+00}  PortSynchronicities={'auto'; 'auto'; 'auto'; 'auto'}  PortSignalSizes={0.000000000000000000e+00; 0.000000000000000000e+00; 0.000000000000000000e+00; 8.000000000000000000e+00}  ClassTemplateSpecKind=implicit  ClassTemplateParamNames={'NSamples'; 'ShiftAcc'; 'DiscardSample'; 'SwapRead'}  ClassTemplateParamKinds={'nontype'; 'nontype'; 'nontype'; 'nontype'}  ClassTemplateParamTypes={'int'; 'int'; 'bool'; 'bool'}  ClassTemplateParamValues={'512', '15', '1', '0'}  ClassCtorParamNames={'taps'}  ClassCtorParamSerializedTypes={'{R{Q1{C{Scint16}4}}}'}  ClassCtorParamValues={'[146-91i 4086+5221i 237-54i -83-21i]'}  ClassIndex=1  ClassCtorIndex=1  ClassTabVisible=on  ClassTemplateParamsVisible=on  ClassCtorDeclVisible=on  ClassCtorParamsVisible=on  FunctionTabVisible=on  FunctionDecl=|  PortAttrs={ 'input', 'sin1', 'input_stream_cint16 * restrict', '', '', '', ''; 'input', 'sin2', 'input_stream_cint16 * restrict', '', '', '', ''; 'input', 'cin', 'input_stream< cacc48_t > *', '', '', '', ''; 'output', 'cout', 'output_stream< cacc48_t > *', '', '', '', 'OUTPUT_SIZE' }  PortAttrsEnables={'off', 'off', 'off', 'off', 'off', 'off', 'off';'off', 'off', 'off', 'off', 'off', 'off', 'off';'off', 'off', 'off', 'off', 'off', 'off', 'off';'off', 'off', 'off', 'off', 'off', 'off', 'on'}  SampleTime=-1  ClassDeclTypeOptions=|  ClassDecl=|  ClassTemplateParams={ 'NSamples', 'int', 'BURST_LENGTH'; 'ShiftAcc', 'int', 'SHIFT_ACC'; 'DiscardSample', 'bool', 'TRUE'; 'SwapRead', 'bool', 'FALSE' }  ClassTemplateParamsEnables={'off', 'off', 'on';'off', 'off', 'on';'off', 'off', 'on';'off', 'off', 'on'}  ClassCtorDeclTypeOptions=C[1 1]@t54@FIR_MultiKernel_cincout(cint16 const ( & taps ) [ 4 ])  ClassCtorDecl=FIR_MultiKernel_cincout(cint16 const ( & taps ) [ 4 ])  ClassCtorParams={ 'taps', 'cint16 const ( &) [ 4 ]', 'phi_6' }  KernelHeaderFile=FirDoubleStream.h  KernelClassName=DoubleStream::FIR_MultiKernel_cincout  KernelFunction=filter  KernelSourceFile=FirDoubleStream.cpp  KernelSearchPaths={'$SRC/aie_kernels'}  PreProcOptions={}  CoreRuntimeRatio=0.9  KernelLocSpec=off  ColRowLocation=[0 0]  blockJsonConstraints="{\"type\":\"constraint\",\"constraintType\":\"coreUtilization\",\"sid\":\"52\",\"lhs\":{\"type\":\"runtimeRatio\",\"args\":{\"type\":\"kernel\",\"name\":\"DualStreamSSR_1/Subsystem/filter33\",\"sid\":\"52\"}},\"rhs\":{\"type\":\"evaluable\",\"expr\":\"0.9\",\"value\":0.9},\"equality\":true}"  deprecateConstraints=1
      KernelAllAttrs=|
      | s[12;12;9;9;19;14;21;23;24;21;12;24;26;26;26;27;28;9;21;23;23;23;24;25;14;19;19;29]@FunctionNameDeclFileNamePortNamesPortTypesPortSerializedTypesPortDirectionsPortWindowSizeEnablesPortWindowMarginEnablesPortSynchronicityEnablesPortSignalSizeEnablesFunctionDeclFunctionTemplateSpecKindFunctionTemplateParamNamesFunctionTemplateParamKindsFunctionTemplateParamTypesFunctionTemplateParamValuesFunctionTemplateParamEnablesClassDeclClassTemplateSpecKindClassTemplateParamNamesClassTemplateParamKindsClassTemplateParamTypesClassTemplateParamValuesClassTemplateParamEnablesClassCtorDeclsClassCtorParamNamesClassCtorParamTypesClassCtorParamSerializedTypes[1 1]@C[28 1]@t6@filtert42@../../../aie/aie_kernels/FirDoubleStream.hC[4 1]@t4@sin1t4@sin2t3@cint4@coutC[4 1]@t30@input_stream_cint16 * restrictt30@input_stream_cint16 * restrictt26@input_stream< cacc48_t > *t27@output_stream< cacc48_t > *C[4 1]@t37@{Q2{P{Tinput_stream{1{t{Scint16}}}}}}t37@{Q2{P{Tinput_stream{1{t{Scint16}}}}}}t35@{P{Tinput_stream{1{t{Scacc48_t}}}}}t36@{P{Toutput_stream{1{t{Scacc48_t}}}}}C[4 1]@t5@inputt5@inputt5@inputt6@outputC[4 1]@l0@l0@l0@l0@C[4 1]@l0@l0@l0@l0@C[4 1]@l0@l0@l0@l0@C[4 1]@l0@l0@l0@l1@t281@namespace DoubleStream {
      | template < int NSamples, int ShiftAcc, bool DiscardSample, bool SwapRead > 
      | void FIR_MultiKernel_cincout::
      | filter(input_stream_cint16 * restrict sin1, input_stream_cint16 * restrict sin2, input_stream< cacc48_t > * cin, output_stream< cacc48_t > * cout);
      | }t4@nonee[0 1]@e[0 1]@e[0 1]@e[0 1]@e[0 1]@t132@namespace DoubleStream {
      | template < int NSamples, int ShiftAcc, bool DiscardSample, bool SwapRead > class FIR_MultiKernel_cincout;
      | }t8@implicitC[4 1]@t8@NSamplest8@ShiftAcct13@DiscardSamplet8@SwapReadC[4 1]@t7@nontypet7@nontypet7@nontypet7@nontypeC[4 1]@t3@intt3@intt4@boolt4@boolC[4 1]@nnnnC[4 1]@l1@l1@l1@l1@C[1 1]@t54@FIR_MultiKernel_cincout(cint16 const ( & taps ) [ 4 ])C[1 1]@C[1 1]@t4@tapsC[1 1]@C[1 1]@t23@cint16 const ( &) [ 4 ]C[1 1]@C[1 1]@t20@{R{Q1{C{Scint16}4}}}
      FunctionDecl=|
      | namespace DoubleStream {
      | template < int NSamples, int ShiftAcc, bool DiscardSample, bool SwapRead > 
      | void FIR_MultiKernel_cincout::
      | filter(input_stream_cint16 * restrict sin1, input_stream_cint16 * restrict sin2, input_stream< cacc48_t > * cin, output_stream< cacc48_t > * cout);
      | }
      ClassDeclTypeOptions=|
      | C[1 1]@t132@namespace DoubleStream {
      | template < int NSamples, int ShiftAcc, bool DiscardSample, bool SwapRead > class FIR_MultiKernel_cincout;
      | }
      ClassDecl=|
      | namespace DoubleStream {
      | template < int NSamples, int ShiftAcc, bool DiscardSample, bool SwapRead > class FIR_MultiKernel_cincout;
      | }
  filter45 : ModelComposer/AIE Class Kernel  KernelAllAttrs=|  PortNames={'sin1'; 'sin2'; 'cin'; 'cout'}  PortSerializedTypes={'{Q2{P{Tinput_stream{1{t{Scint16}}}}}}'; '{Q2{P{Tinput_stream{1{t{Scint16}}}}}}'; '{P{Tinput_stream{1{t{Scacc48_t}}}}}'; '{P{Toutput_stream{1{t{Scacc48_t}}}}}'}  PortWindowSizes={0.000000000000000000e+00; 0.000000000000000000e+00; 0.000000000000000000e+00; 0.000000000000000000e+00}  PortWindowMargins={0.000000000000000000e+00; 0.000000000000000000e+00; 0.000000000000000000e+00; 0.000000000000000000e+00}  PortSynchronicities={'auto'; 'auto'; 'auto'; 'auto'}  PortSignalSizes={0.000000000000000000e+00; 0.000000000000000000e+00; 0.000000000000000000e+00; 8.000000000000000000e+00}  ClassTemplateSpecKind=implicit  ClassTemplateParamNames={'NSamples'; 'ShiftAcc'; 'DiscardSample'; 'SwapRead'}  ClassTemplateParamKinds={'nontype'; 'nontype'; 'nontype'; 'nontype'}  ClassTemplateParamTypes={'int'; 'int'; 'bool'; 'bool'}  ClassTemplateParamValues={'512', '15', '1', '0'}  ClassCtorParamNames={'taps'}  ClassCtorParamSerializedTypes={'{R{Q1{C{Scint16}4}}}'}  ClassCtorParamValues={'[146-91i 4086+5221i 237-54i -83-21i]'}  ClassIndex=1  ClassCtorIndex=1  ClassTabVisible=on  ClassTemplateParamsVisible=on  ClassCtorDeclVisible=on  ClassCtorParamsVisible=on  FunctionTabVisible=on  FunctionDecl=|  PortAttrs={ 'input', 'sin1', 'input_stream_cint16 * restrict', '', '', '', ''; 'input', 'sin2', 'input_stream_cint16 * restrict', '', '', '', ''; 'input', 'cin', 'input_stream< cacc48_t > *', '', '', '', ''; 'output', 'cout', 'output_stream< cacc48_t > *', '', '', '', 'OUTPUT_SIZE' }  PortAttrsEnables={'off', 'off', 'off', 'off', 'off', 'off', 'off';'off', 'off', 'off', 'off', 'off', 'off', 'off';'off', 'off', 'off', 'off', 'off', 'off', 'off';'off', 'off', 'off', 'off', 'off', 'off', 'on'}  SampleTime=-1  ClassDeclTypeOptions=|  ClassDecl=|  ClassTemplateParams={ 'NSamples', 'int', 'BURST_LENGTH'; 'ShiftAcc', 'int', 'SHIFT_ACC'; 'DiscardSample', 'bool', 'TRUE'; 'SwapRead', 'bool', 'FALSE' }  ClassTemplateParamsEnables={'off', 'off', 'on';'off', 'off', 'on';'off', 'off', 'on';'off', 'off', 'on'}  ClassCtorDeclTypeOptions=C[1 1]@t54@FIR_MultiKernel_cincout(cint16 const ( & taps ) [ 4 ])  ClassCtorDecl=FIR_MultiKernel_cincout(cint16 const ( & taps ) [ 4 ])  ClassCtorParams={ 'taps', 'cint16 const ( &) [ 4 ]', 'phi_6' }  KernelHeaderFile=FirDoubleStream.h  KernelClassName=DoubleStream::FIR_MultiKernel_cincout  KernelFunction=filter  KernelSourceFile=FirDoubleStream.cpp  KernelSearchPaths={'$SRC/aie_kernels'}  PreProcOptions={}  CoreRuntimeRatio=0.9  KernelLocSpec=off  ColRowLocation=[0 0]  blockJsonConstraints="{\"type\":\"constraint\",\"constraintType\":\"coreUtilization\",\"sid\":\"65\",\"lhs\":{\"type\":\"runtimeRatio\",\"args\":{\"type\":\"kernel\",\"name\":\"DualStreamSSR_1/Subsystem/filter46\",\"sid\":\"65\"}},\"rhs\":{\"type\":\"evaluable\",\"expr\":\"0.9\",\"value\":0.9},\"equality\":true}"  deprecateConstraints=1
      KernelAllAttrs=|
      | s[12;12;9;9;19;14;21;23;24;21;12;24;26;26;26;27;28;9;21;23;23;23;24;25;14;19;19;29]@FunctionNameDeclFileNamePortNamesPortTypesPortSerializedTypesPortDirectionsPortWindowSizeEnablesPortWindowMarginEnablesPortSynchronicityEnablesPortSignalSizeEnablesFunctionDeclFunctionTemplateSpecKindFunctionTemplateParamNamesFunctionTemplateParamKindsFunctionTemplateParamTypesFunctionTemplateParamValuesFunctionTemplateParamEnablesClassDeclClassTemplateSpecKindClassTemplateParamNamesClassTemplateParamKindsClassTemplateParamTypesClassTemplateParamValuesClassTemplateParamEnablesClassCtorDeclsClassCtorParamNamesClassCtorParamTypesClassCtorParamSerializedTypes[1 1]@C[28 1]@t6@filtert42@../../../aie/aie_kernels/FirDoubleStream.hC[4 1]@t4@sin1t4@sin2t3@cint4@coutC[4 1]@t30@input_stream_cint16 * restrictt30@input_stream_cint16 * restrictt26@input_stream< cacc48_t > *t27@output_stream< cacc48_t > *C[4 1]@t37@{Q2{P{Tinput_stream{1{t{Scint16}}}}}}t37@{Q2{P{Tinput_stream{1{t{Scint16}}}}}}t35@{P{Tinput_stream{1{t{Scacc48_t}}}}}t36@{P{Toutput_stream{1{t{Scacc48_t}}}}}C[4 1]@t5@inputt5@inputt5@inputt6@outputC[4 1]@l0@l0@l0@l0@C[4 1]@l0@l0@l0@l0@C[4 1]@l0@l0@l0@l0@C[4 1]@l0@l0@l0@l1@t281@namespace DoubleStream {
      | template < int NSamples, int ShiftAcc, bool DiscardSample, bool SwapRead > 
      | void FIR_MultiKernel_cincout::
      | filter(input_stream_cint16 * restrict sin1, input_stream_cint16 * restrict sin2, input_stream< cacc48_t > * cin, output_stream< cacc48_t > * cout);
      | }t4@nonee[0 1]@e[0 1]@e[0 1]@e[0 1]@e[0 1]@t132@namespace DoubleStream {
      | template < int NSamples, int ShiftAcc, bool DiscardSample, bool SwapRead > class FIR_MultiKernel_cincout;
      | }t8@implicitC[4 1]@t8@NSamplest8@ShiftAcct13@DiscardSamplet8@SwapReadC[4 1]@t7@nontypet7@nontypet7@nontypet7@nontypeC[4 1]@t3@intt3@intt4@boolt4@boolC[4 1]@nnnnC[4 1]@l1@l1@l1@l1@C[1 1]@t54@FIR_MultiKernel_cincout(cint16 const ( & taps ) [ 4 ])C[1 1]@C[1 1]@t4@tapsC[1 1]@C[1 1]@t23@cint16 const ( &) [ 4 ]C[1 1]@C[1 1]@t20@{R{Q1{C{Scint16}4}}}
      FunctionDecl=|
      | namespace DoubleStream {
      | template < int NSamples, int ShiftAcc, bool DiscardSample, bool SwapRead > 
      | void FIR_MultiKernel_cincout::
      | filter(input_stream_cint16 * restrict sin1, input_stream_cint16 * restrict sin2, input_stream< cacc48_t > * cin, output_stream< cacc48_t > * cout);
      | }
      ClassDeclTypeOptions=|
      | C[1 1]@t132@namespace DoubleStream {
      | template < int NSamples, int ShiftAcc, bool DiscardSample, bool SwapRead > class FIR_MultiKernel_cincout;
      | }
      ClassDecl=|
      | namespace DoubleStream {
      | template < int NSamples, int ShiftAcc, bool DiscardSample, bool SwapRead > class FIR_MultiKernel_cincout;
      | }
  filter46 : ModelComposer/AIE Class Kernel  KernelAllAttrs=|  PortNames={'sin1'; 'sin2'; 'cin'; 'cout'}  PortSerializedTypes={'{Q2{P{Tinput_stream{1{t{Scint16}}}}}}'; '{Q2{P{Tinput_stream{1{t{Scint16}}}}}}'; '{P{Tinput_stream{1{t{Scacc48_t}}}}}'; '{P{Toutput_stream{1{t{Scacc48_t}}}}}'}  PortWindowSizes={0.000000000000000000e+00; 0.000000000000000000e+00; 0.000000000000000000e+00; 0.000000000000000000e+00}  PortWindowMargins={0.000000000000000000e+00; 0.000000000000000000e+00; 0.000000000000000000e+00; 0.000000000000000000e+00}  PortSynchronicities={'auto'; 'auto'; 'auto'; 'auto'}  PortSignalSizes={0.000000000000000000e+00; 0.000000000000000000e+00; 0.000000000000000000e+00; 8.000000000000000000e+00}  ClassTemplateSpecKind=implicit  ClassTemplateParamNames={'NSamples'; 'ShiftAcc'; 'DiscardSample'; 'SwapRead'}  ClassTemplateParamKinds={'nontype'; 'nontype'; 'nontype'; 'nontype'}  ClassTemplateParamTypes={'int'; 'int'; 'bool'; 'bool'}  ClassTemplateParamValues={'512', '15', '1', '0'}  ClassCtorParamNames={'taps'}  ClassCtorParamSerializedTypes={'{R{Q1{C{Scint16}4}}}'}  ClassCtorParamValues={'[14-121i 1454-497i 237+96i -121+233i]'}  ClassIndex=1  ClassCtorIndex=1  ClassTabVisible=on  ClassTemplateParamsVisible=on  ClassCtorDeclVisible=on  ClassCtorParamsVisible=on  FunctionTabVisible=on  FunctionDecl=|  PortAttrs={ 'input', 'sin1', 'input_stream_cint16 * restrict', '', '', '', ''; 'input', 'sin2', 'input_stream_cint16 * restrict', '', '', '', ''; 'input', 'cin', 'input_stream< cacc48_t > *', '', '', '', ''; 'output', 'cout', 'output_stream< cacc48_t > *', '', '', '', 'OUTPUT_SIZE' }  PortAttrsEnables={'off', 'off', 'off', 'off', 'off', 'off', 'off';'off', 'off', 'off', 'off', 'off', 'off', 'off';'off', 'off', 'off', 'off', 'off', 'off', 'off';'off', 'off', 'off', 'off', 'off', 'off', 'on'}  SampleTime=-1  ClassDeclTypeOptions=|  ClassDecl=|  ClassTemplateParams={ 'NSamples', 'int', 'BURST_LENGTH'; 'ShiftAcc', 'int', 'SHIFT_ACC'; 'DiscardSample', 'bool', 'TRUE'; 'SwapRead', 'bool', 'FALSE' }  ClassTemplateParamsEnables={'off', 'off', 'on';'off', 'off', 'on';'off', 'off', 'on';'off', 'off', 'on'}  ClassCtorDeclTypeOptions=C[1 1]@t54@FIR_MultiKernel_cincout(cint16 const ( & taps ) [ 4 ])  ClassCtorDecl=FIR_MultiKernel_cincout(cint16 const ( & taps ) [ 4 ])  ClassCtorParams={ 'taps', 'cint16 const ( &) [ 4 ]', 'phi_3' }  KernelHeaderFile=FirDoubleStream.h  KernelClassName=DoubleStream::FIR_MultiKernel_cincout  KernelFunction=filter  KernelSourceFile=FirDoubleStream.cpp  KernelSearchPaths={'$SRC/aie_kernels'}  PreProcOptions={}  CoreRuntimeRatio=0.9  KernelLocSpec=off  ColRowLocation=[0 0]  blockJsonConstraints="{\"type\":\"constraint\",\"constraintType\":\"coreUtilization\",\"sid\":\"65\",\"lhs\":{\"type\":\"runtimeRatio\",\"args\":{\"type\":\"kernel\",\"name\":\"DualStreamSSR_1/Subsystem/filter46\",\"sid\":\"65\"}},\"rhs\":{\"type\":\"evaluable\",\"expr\":\"0.9\",\"value\":0.9},\"equality\":true}"  deprecateConstraints=1
      KernelAllAttrs=|
      | s[12;12;9;9;19;14;21;23;24;21;12;24;26;26;26;27;28;9;21;23;23;23;24;25;14;19;19;29]@FunctionNameDeclFileNamePortNamesPortTypesPortSerializedTypesPortDirectionsPortWindowSizeEnablesPortWindowMarginEnablesPortSynchronicityEnablesPortSignalSizeEnablesFunctionDeclFunctionTemplateSpecKindFunctionTemplateParamNamesFunctionTemplateParamKindsFunctionTemplateParamTypesFunctionTemplateParamValuesFunctionTemplateParamEnablesClassDeclClassTemplateSpecKindClassTemplateParamNamesClassTemplateParamKindsClassTemplateParamTypesClassTemplateParamValuesClassTemplateParamEnablesClassCtorDeclsClassCtorParamNamesClassCtorParamTypesClassCtorParamSerializedTypes[1 1]@C[28 1]@t6@filtert42@../../../aie/aie_kernels/FirDoubleStream.hC[4 1]@t4@sin1t4@sin2t3@cint4@coutC[4 1]@t30@input_stream_cint16 * restrictt30@input_stream_cint16 * restrictt26@input_stream< cacc48_t > *t27@output_stream< cacc48_t > *C[4 1]@t37@{Q2{P{Tinput_stream{1{t{Scint16}}}}}}t37@{Q2{P{Tinput_stream{1{t{Scint16}}}}}}t35@{P{Tinput_stream{1{t{Scacc48_t}}}}}t36@{P{Toutput_stream{1{t{Scacc48_t}}}}}C[4 1]@t5@inputt5@inputt5@inputt6@outputC[4 1]@l0@l0@l0@l0@C[4 1]@l0@l0@l0@l0@C[4 1]@l0@l0@l0@l0@C[4 1]@l0@l0@l0@l1@t281@namespace DoubleStream {
      | template < int NSamples, int ShiftAcc, bool DiscardSample, bool SwapRead > 
      | void FIR_MultiKernel_cincout::
      | filter(input_stream_cint16 * restrict sin1, input_stream_cint16 * restrict sin2, input_stream< cacc48_t > * cin, output_stream< cacc48_t > * cout);
      | }t4@nonee[0 1]@e[0 1]@e[0 1]@e[0 1]@e[0 1]@t132@namespace DoubleStream {
      | template < int NSamples, int ShiftAcc, bool DiscardSample, bool SwapRead > class FIR_MultiKernel_cincout;
      | }t8@implicitC[4 1]@t8@NSamplest8@ShiftAcct13@DiscardSamplet8@SwapReadC[4 1]@t7@nontypet7@nontypet7@nontypet7@nontypeC[4 1]@t3@intt3@intt4@boolt4@boolC[4 1]@nnnnC[4 1]@l1@l1@l1@l1@C[1 1]@t54@FIR_MultiKernel_cincout(cint16 const ( & taps ) [ 4 ])C[1 1]@C[1 1]@t4@tapsC[1 1]@C[1 1]@t23@cint16 const ( &) [ 4 ]C[1 1]@C[1 1]@t20@{R{Q1{C{Scint16}4}}}
      FunctionDecl=|
      | namespace DoubleStream {
      | template < int NSamples, int ShiftAcc, bool DiscardSample, bool SwapRead > 
      | void FIR_MultiKernel_cincout::
      | filter(input_stream_cint16 * restrict sin1, input_stream_cint16 * restrict sin2, input_stream< cacc48_t > * cin, output_stream< cacc48_t > * cout);
      | }
      ClassDeclTypeOptions=|
      | C[1 1]@t132@namespace DoubleStream {
      | template < int NSamples, int ShiftAcc, bool DiscardSample, bool SwapRead > class FIR_MultiKernel_cincout;
      | }
      ClassDecl=|
      | namespace DoubleStream {
      | template < int NSamples, int ShiftAcc, bool DiscardSample, bool SwapRead > class FIR_MultiKernel_cincout;
      | }
  filter47 : ModelComposer/AIE Class Kernel  KernelAllAttrs=|  PortNames={'sin1'; 'sin2'; 'cin'; 'cout'}  PortSerializedTypes={'{Q2{P{Tinput_stream{1{t{Scint16}}}}}}'; '{Q2{P{Tinput_stream{1{t{Scint16}}}}}}'; '{P{Tinput_stream{1{t{Scacc48_t}}}}}'; '{P{Toutput_stream{1{t{Scacc48_t}}}}}'}  PortWindowSizes={0.000000000000000000e+00; 0.000000000000000000e+00; 0.000000000000000000e+00; 0.000000000000000000e+00}  PortWindowMargins={0.000000000000000000e+00; 0.000000000000000000e+00; 0.000000000000000000e+00; 0.000000000000000000e+00}  PortSynchronicities={'auto'; 'auto'; 'auto'; 'auto'}  PortSignalSizes={0.000000000000000000e+00; 0.000000000000000000e+00; 0.000000000000000000e+00; 8.000000000000000000e+00}  ClassTemplateSpecKind=implicit  ClassTemplateParamNames={'NSamples'; 'ShiftAcc'; 'DiscardSample'; 'SwapRead'}  ClassTemplateParamKinds={'nontype'; 'nontype'; 'nontype'; 'nontype'}  ClassTemplateParamTypes={'int'; 'int'; 'bool'; 'bool'}  ClassTemplateParamValues={'512', '15', '1', '0'}  ClassCtorParamNames={'taps'}  ClassCtorParamSerializedTypes={'{R{Q1{C{Scint16}4}}}'}  ClassCtorParamValues={'[-21+26i 1183+239i 248-2878i -160+111i]'}  ClassIndex=1  ClassCtorIndex=1  ClassTabVisible=on  ClassTemplateParamsVisible=on  ClassCtorDeclVisible=on  ClassCtorParamsVisible=on  FunctionTabVisible=on  FunctionDecl=|  PortAttrs={ 'input', 'sin1', 'input_stream_cint16 * restrict', '', '', '', ''; 'input', 'sin2', 'input_stream_cint16 * restrict', '', '', '', ''; 'input', 'cin', 'input_stream< cacc48_t > *', '', '', '', ''; 'output', 'cout', 'output_stream< cacc48_t > *', '', '', '', 'OUTPUT_SIZE' }  PortAttrsEnables={'off', 'off', 'off', 'off', 'off', 'off', 'off';'off', 'off', 'off', 'off', 'off', 'off', 'off';'off', 'off', 'off', 'off', 'off', 'off', 'off';'off', 'off', 'off', 'off', 'off', 'off', 'on'}  SampleTime=-1  ClassDeclTypeOptions=|  ClassDecl=|  ClassTemplateParams={ 'NSamples', 'int', 'BURST_LENGTH'; 'ShiftAcc', 'int', 'SHIFT_ACC'; 'DiscardSample', 'bool', 'TRUE'; 'SwapRead', 'bool', 'FALSE' }  ClassTemplateParamsEnables={'off', 'off', 'on';'off', 'off', 'on';'off', 'off', 'on';'off', 'off', 'on'}  ClassCtorDeclTypeOptions=C[1 1]@t54@FIR_MultiKernel_cincout(cint16 const ( & taps ) [ 4 ])  ClassCtorDecl=FIR_MultiKernel_cincout(cint16 const ( & taps ) [ 4 ])  ClassCtorParams={ 'taps', 'cint16 const ( &) [ 4 ]', 'phi_2' }  KernelHeaderFile=FirDoubleStream.h  KernelClassName=DoubleStream::FIR_MultiKernel_cincout  KernelFunction=filter  KernelSourceFile=FirDoubleStream.cpp  KernelSearchPaths={'$SRC/aie_kernels'}  PreProcOptions={}  CoreRuntimeRatio=0.9  KernelLocSpec=off  ColRowLocation=[0 0]  blockJsonConstraints="{\"type\":\"constraint\",\"constraintType\":\"coreUtilization\",\"sid\":\"66\",\"lhs\":{\"type\":\"runtimeRatio\",\"args\":{\"type\":\"kernel\",\"name\":\"DualStreamSSR_1/Subsystem/filter47\",\"sid\":\"66\"}},\"rhs\":{\"type\":\"evaluable\",\"expr\":\"0.9\",\"value\":0.9},\"equality\":true}"  deprecateConstraints=1
      KernelAllAttrs=|
      | s[12;12;9;9;19;14;21;23;24;21;12;24;26;26;26;27;28;9;21;23;23;23;24;25;14;19;19;29]@FunctionNameDeclFileNamePortNamesPortTypesPortSerializedTypesPortDirectionsPortWindowSizeEnablesPortWindowMarginEnablesPortSynchronicityEnablesPortSignalSizeEnablesFunctionDeclFunctionTemplateSpecKindFunctionTemplateParamNamesFunctionTemplateParamKindsFunctionTemplateParamTypesFunctionTemplateParamValuesFunctionTemplateParamEnablesClassDeclClassTemplateSpecKindClassTemplateParamNamesClassTemplateParamKindsClassTemplateParamTypesClassTemplateParamValuesClassTemplateParamEnablesClassCtorDeclsClassCtorParamNamesClassCtorParamTypesClassCtorParamSerializedTypes[1 1]@C[28 1]@t6@filtert42@../../../aie/aie_kernels/FirDoubleStream.hC[4 1]@t4@sin1t4@sin2t3@cint4@coutC[4 1]@t30@input_stream_cint16 * restrictt30@input_stream_cint16 * restrictt26@input_stream< cacc48_t > *t27@output_stream< cacc48_t > *C[4 1]@t37@{Q2{P{Tinput_stream{1{t{Scint16}}}}}}t37@{Q2{P{Tinput_stream{1{t{Scint16}}}}}}t35@{P{Tinput_stream{1{t{Scacc48_t}}}}}t36@{P{Toutput_stream{1{t{Scacc48_t}}}}}C[4 1]@t5@inputt5@inputt5@inputt6@outputC[4 1]@l0@l0@l0@l0@C[4 1]@l0@l0@l0@l0@C[4 1]@l0@l0@l0@l0@C[4 1]@l0@l0@l0@l1@t281@namespace DoubleStream {
      | template < int NSamples, int ShiftAcc, bool DiscardSample, bool SwapRead > 
      | void FIR_MultiKernel_cincout::
      | filter(input_stream_cint16 * restrict sin1, input_stream_cint16 * restrict sin2, input_stream< cacc48_t > * cin, output_stream< cacc48_t > * cout);
      | }t4@nonee[0 1]@e[0 1]@e[0 1]@e[0 1]@e[0 1]@t132@namespace DoubleStream {
      | template < int NSamples, int ShiftAcc, bool DiscardSample, bool SwapRead > class FIR_MultiKernel_cincout;
      | }t8@implicitC[4 1]@t8@NSamplest8@ShiftAcct13@DiscardSamplet8@SwapReadC[4 1]@t7@nontypet7@nontypet7@nontypet7@nontypeC[4 1]@t3@intt3@intt4@boolt4@boolC[4 1]@nnnnC[4 1]@l1@l1@l1@l1@C[1 1]@t54@FIR_MultiKernel_cincout(cint16 const ( & taps ) [ 4 ])C[1 1]@C[1 1]@t4@tapsC[1 1]@C[1 1]@t23@cint16 const ( &) [ 4 ]C[1 1]@C[1 1]@t20@{R{Q1{C{Scint16}4}}}
      FunctionDecl=|
      | namespace DoubleStream {
      | template < int NSamples, int ShiftAcc, bool DiscardSample, bool SwapRead > 
      | void FIR_MultiKernel_cincout::
      | filter(input_stream_cint16 * restrict sin1, input_stream_cint16 * restrict sin2, input_stream< cacc48_t > * cin, output_stream< cacc48_t > * cout);
      | }
      ClassDeclTypeOptions=|
      | C[1 1]@t132@namespace DoubleStream {
      | template < int NSamples, int ShiftAcc, bool DiscardSample, bool SwapRead > class FIR_MultiKernel_cincout;
      | }
      ClassDecl=|
      | namespace DoubleStream {
      | template < int NSamples, int ShiftAcc, bool DiscardSample, bool SwapRead > class FIR_MultiKernel_cincout;
      | }
  filter48 : ModelComposer/AIE Class Kernel  KernelAllAttrs=|  PortNames={'sin1'; 'sin2'; 'cin'; 'sout1'; 'sout2'}  PortSerializedTypes={'{Q2{P{Tinput_stream{1{t{Scint16}}}}}}'; '{Q2{P{Tinput_stream{1{t{Scint16}}}}}}'; '{P{Tinput_stream{1{t{Scacc48_t}}}}}'; '{Q2{P{Toutput_stream{1{t{Scint16}}}}}}'; '{Q2{P{Toutput_stream{1{t{Scint16}}}}}}'}  PortWindowSizes={0.000000000000000000e+00; 0.000000000000000000e+00; 0.000000000000000000e+00; 0.000000000000000000e+00; 0.000000000000000000e+00}  PortWindowMargins={0.000000000000000000e+00; 0.000000000000000000e+00; 0.000000000000000000e+00; 0.000000000000000000e+00; 0.000000000000000000e+00}  PortSynchronicities={'auto'; 'auto'; 'auto'; 'auto'; 'auto'}  PortSignalSizes={0.000000000000000000e+00; 0.000000000000000000e+00; 0.000000000000000000e+00; 4.000000000000000000e+00; 4.000000000000000000e+00}  ClassTemplateSpecKind=implicit  ClassTemplateParamNames={'NSamples'; 'ShiftAcc'; 'DiscardSample'; 'SwapRead'}  ClassTemplateParamKinds={'nontype'; 'nontype'; 'nontype'; 'nontype'}  ClassTemplateParamTypes={'int'; 'int'; 'bool'; 'bool'}  ClassTemplateParamValues={'512', '15', '1', '0'}  ClassCtorParamNames={'taps'}  ClassCtorParamSerializedTypes={'{R{Q1{C{Scint16}4}}}'}  ClassCtorParamValues={'[-83+21i 237+54i 4086-5221i 146+91i]'}  ClassIndex=1  ClassCtorIndex=1  ClassTabVisible=on  ClassTemplateParamsVisible=on  ClassCtorDeclVisible=on  ClassCtorParamsVisible=on  FunctionTabVisible=on  FunctionDecl=|  PortAttrs={ 'input', 'sin1', 'input_stream_cint16 * restrict', '', '', '', ''; 'input', 'sin2', 'input_stream_cint16 * restrict', '', '', '', ''; 'input', 'cin', 'input_stream< cacc48_t > *', '', '', '', ''; 'output', 'sout1', 'output_stream_cint16 * restrict', '', '', '', 'OUTPUT_SIZE/2'; 'output', 'sout2', 'output_stream_cint16 * restrict', '', '', '', 'OUTPUT_SIZE/2' }  PortAttrsEnables={'off', 'off', 'off', 'off', 'off', 'off', 'off';'off', 'off', 'off', 'off', 'off', 'off', 'off';'off', 'off', 'off', 'off', 'off', 'off', 'off';'off', 'off', 'off', 'off', 'off', 'off', 'on';'off', 'off', 'off', 'off', 'off', 'off', 'on'}  SampleTime=-1  ClassDeclTypeOptions=|  ClassDecl=|  ClassTemplateParams={ 'NSamples', 'int', 'BURST_LENGTH'; 'ShiftAcc', 'int', 'SHIFT_ACC'; 'DiscardSample', 'bool', 'TRUE'; 'SwapRead', 'bool', 'FALSE' }  ClassTemplateParamsEnables={'off', 'off', 'on';'off', 'off', 'on';'off', 'off', 'on';'off', 'off', 'on'}  ClassCtorDeclTypeOptions=C[1 1]@t50@FIR_MultiKernel_cin(cint16 const ( & taps ) [ 4 ])  ClassCtorDecl=FIR_MultiKernel_cin(cint16 const ( & taps ) [ 4 ])  ClassCtorParams={ 'taps', 'cint16 const ( &) [ 4 ]', 'phi_1' }  KernelHeaderFile=FirDoubleStream.h  KernelClassName=DoubleStream::FIR_MultiKernel_cin  KernelFunction=filter  KernelSourceFile=FirDoubleStream.cpp  KernelSearchPaths={'$SRC/aie_kernels'}  PreProcOptions={}  CoreRuntimeRatio=0.9  KernelLocSpec=off  ColRowLocation=[0 0]  blockJsonConstraints="{\"type\":\"constraint\",\"constraintType\":\"coreUtilization\",\"sid\":\"67\",\"lhs\":{\"type\":\"runtimeRatio\",\"args\":{\"type\":\"kernel\",\"name\":\"DualStreamSSR_1/Subsystem/filter48\",\"sid\":\"67\"}},\"rhs\":{\"type\":\"evaluable\",\"expr\":\"0.9\",\"value\":0.9},\"equality\":true}"  deprecateConstraints=1
      KernelAllAttrs=|
      | s[12;12;9;9;19;14;21;23;24;21;12;24;26;26;26;27;28;9;21;23;23;23;24;25;14;19;19;29]@FunctionNameDeclFileNamePortNamesPortTypesPortSerializedTypesPortDirectionsPortWindowSizeEnablesPortWindowMarginEnablesPortSynchronicityEnablesPortSignalSizeEnablesFunctionDeclFunctionTemplateSpecKindFunctionTemplateParamNamesFunctionTemplateParamKindsFunctionTemplateParamTypesFunctionTemplateParamValuesFunctionTemplateParamEnablesClassDeclClassTemplateSpecKindClassTemplateParamNamesClassTemplateParamKindsClassTemplateParamTypesClassTemplateParamValuesClassTemplateParamEnablesClassCtorDeclsClassCtorParamNamesClassCtorParamTypesClassCtorParamSerializedTypes[1 1]@C[28 1]@t6@filtert42@../../../aie/aie_kernels/FirDoubleStream.hC[5 1]@t4@sin1t4@sin2t3@cint5@sout1t5@sout2C[5 1]@t30@input_stream_cint16 * restrictt30@input_stream_cint16 * restrictt26@input_stream< cacc48_t > *t31@output_stream_cint16 * restrictt31@output_stream_cint16 * restrictC[5 1]@t37@{Q2{P{Tinput_stream{1{t{Scint16}}}}}}t37@{Q2{P{Tinput_stream{1{t{Scint16}}}}}}t35@{P{Tinput_stream{1{t{Scacc48_t}}}}}t38@{Q2{P{Toutput_stream{1{t{Scint16}}}}}}t38@{Q2{P{Toutput_stream{1{t{Scint16}}}}}}C[5 1]@t5@inputt5@inputt5@inputt6@outputt6@outputC[5 1]@l0@l0@l0@l0@l0@C[5 1]@l0@l0@l0@l0@l0@C[5 1]@l0@l0@l0@l0@l0@C[5 1]@l0@l0@l0@l1@l1@t321@namespace DoubleStream {
      | template < int NSamples, int ShiftAcc, bool DiscardSample, bool SwapRead > 
      | void FIR_MultiKernel_cin::
      | filter(input_stream_cint16 * restrict sin1, input_stream_cint16 * restrict sin2, input_stream< cacc48_t > * cin, output_stream_cint16 * restrict sout1, output_stream_cint16 * restrict sout2);
      | }t4@nonee[0 1]@e[0 1]@e[0 1]@e[0 1]@e[0 1]@t128@namespace DoubleStream {
      | template < int NSamples, int ShiftAcc, bool DiscardSample, bool SwapRead > class FIR_MultiKernel_cin;
      | }t8@implicitC[4 1]@t8@NSamplest8@ShiftAcct13@DiscardSamplet8@SwapReadC[4 1]@t7@nontypet7@nontypet7@nontypet7@nontypeC[4 1]@t3@intt3@intt4@boolt4@boolC[4 1]@nnnnC[4 1]@l1@l1@l1@l1@C[1 1]@t50@FIR_MultiKernel_cin(cint16 const ( & taps ) [ 4 ])C[1 1]@C[1 1]@t4@tapsC[1 1]@C[1 1]@t23@cint16 const ( &) [ 4 ]C[1 1]@C[1 1]@t20@{R{Q1{C{Scint16}4}}}
      FunctionDecl=|
      | namespace DoubleStream {
      | template < int NSamples, int ShiftAcc, bool DiscardSample, bool SwapRead > 
      | void FIR_MultiKernel_cin::
      | filter(input_stream_cint16 * restrict sin1, input_stream_cint16 * restrict sin2, input_stream< cacc48_t > * cin, output_stream_cint16 * restrict sout1, output_stream_cint16 * restrict sout2);
      | }
      ClassDeclTypeOptions=|
      | C[1 1]@t128@namespace DoubleStream {
      | template < int NSamples, int ShiftAcc, bool DiscardSample, bool SwapRead > class FIR_MultiKernel_cin;
      | }
      ClassDecl=|
      | namespace DoubleStream {
      | template < int NSamples, int ShiftAcc, bool DiscardSample, bool SwapRead > class FIR_MultiKernel_cin;
      | }
  filter49 : ModelComposer/AIE Class Kernel  KernelAllAttrs=|  PortNames={'sin1'; 'sin2'; 'cin'; 'cout'}  PortSerializedTypes={'{Q2{P{Tinput_stream{1{t{Scint16}}}}}}'; '{Q2{P{Tinput_stream{1{t{Scint16}}}}}}'; '{P{Tinput_stream{1{t{Scacc48_t}}}}}'; '{P{Toutput_stream{1{t{Scacc48_t}}}}}'}  PortWindowSizes={0.000000000000000000e+00; 0.000000000000000000e+00; 0.000000000000000000e+00; 0.000000000000000000e+00}  PortWindowMargins={0.000000000000000000e+00; 0.000000000000000000e+00; 0.000000000000000000e+00; 0.000000000000000000e+00}  PortSynchronicities={'auto'; 'auto'; 'auto'; 'auto'}  PortSignalSizes={0.000000000000000000e+00; 0.000000000000000000e+00; 0.000000000000000000e+00; 8.000000000000000000e+00}  ClassTemplateSpecKind=implicit  ClassTemplateParamNames={'NSamples'; 'ShiftAcc'; 'DiscardSample'; 'SwapRead'}  ClassTemplateParamKinds={'nontype'; 'nontype'; 'nontype'; 'nontype'}  ClassTemplateParamTypes={'int'; 'int'; 'bool'; 'bool'}  ClassTemplateParamValues={'512', '15', '1', '0'}  ClassCtorParamNames={'taps'}  ClassCtorParamSerializedTypes={'{R{Q1{C{Scint16}4}}}'}  ClassCtorParamValues={'[-121-233i 237-96i 1454+497i 14+121i]'}  ClassIndex=1  ClassCtorIndex=1  ClassTabVisible=on  ClassTemplateParamsVisible=on  ClassCtorDeclVisible=on  ClassCtorParamsVisible=on  FunctionTabVisible=on  FunctionDecl=|  PortAttrs={ 'input', 'sin1', 'input_stream_cint16 * restrict', '', '', '', ''; 'input', 'sin2', 'input_stream_cint16 * restrict', '', '', '', ''; 'input', 'cin', 'input_stream< cacc48_t > *', '', '', '', ''; 'output', 'cout', 'output_stream< cacc48_t > *', '', '', '', 'OUTPUT_SIZE' }  PortAttrsEnables={'off', 'off', 'off', 'off', 'off', 'off', 'off';'off', 'off', 'off', 'off', 'off', 'off', 'off';'off', 'off', 'off', 'off', 'off', 'off', 'off';'off', 'off', 'off', 'off', 'off', 'off', 'on'}  SampleTime=-1  ClassDeclTypeOptions=|  ClassDecl=|  ClassTemplateParams={ 'NSamples', 'int', 'BURST_LENGTH'; 'ShiftAcc', 'int', 'SHIFT_ACC'; 'DiscardSample', 'bool', 'TRUE'; 'SwapRead', 'bool', 'FALSE' }  ClassTemplateParamsEnables={'off', 'off', 'on';'off', 'off', 'on';'off', 'off', 'on';'off', 'off', 'on'}  ClassCtorDeclTypeOptions=C[1 1]@t54@FIR_MultiKernel_cincout(cint16 const ( & taps ) [ 4 ])  ClassCtorDecl=FIR_MultiKernel_cincout(cint16 const ( & taps ) [ 4 ])  ClassCtorParams={ 'taps', 'cint16 const ( &) [ 4 ]', 'phi_4' }  KernelHeaderFile=FirDoubleStream.h  KernelClassName=DoubleStream::FIR_MultiKernel_cincout  KernelFunction=filter  KernelSourceFile=FirDoubleStream.cpp  KernelSearchPaths={'$SRC/aie_kernels'}  PreProcOptions={}  CoreRuntimeRatio=0.9  KernelLocSpec=off  ColRowLocation=[0 0]  blockJsonConstraints="{\"type\":\"constraint\",\"constraintType\":\"coreUtilization\",\"sid\":\"60\",\"lhs\":{\"type\":\"runtimeRatio\",\"args\":{\"type\":\"kernel\",\"name\":\"DualStreamSSR_1/Subsystem/filter41\",\"sid\":\"60\"}},\"rhs\":{\"type\":\"evaluable\",\"expr\":\"0.9\",\"value\":0.9},\"equality\":true}"  deprecateConstraints=1
      KernelAllAttrs=|
      | s[12;12;9;9;19;14;21;23;24;21;12;24;26;26;26;27;28;9;21;23;23;23;24;25;14;19;19;29]@FunctionNameDeclFileNamePortNamesPortTypesPortSerializedTypesPortDirectionsPortWindowSizeEnablesPortWindowMarginEnablesPortSynchronicityEnablesPortSignalSizeEnablesFunctionDeclFunctionTemplateSpecKindFunctionTemplateParamNamesFunctionTemplateParamKindsFunctionTemplateParamTypesFunctionTemplateParamValuesFunctionTemplateParamEnablesClassDeclClassTemplateSpecKindClassTemplateParamNamesClassTemplateParamKindsClassTemplateParamTypesClassTemplateParamValuesClassTemplateParamEnablesClassCtorDeclsClassCtorParamNamesClassCtorParamTypesClassCtorParamSerializedTypes[1 1]@C[28 1]@t6@filtert42@../../../aie/aie_kernels/FirDoubleStream.hC[4 1]@t4@sin1t4@sin2t3@cint4@coutC[4 1]@t30@input_stream_cint16 * restrictt30@input_stream_cint16 * restrictt26@input_stream< cacc48_t > *t27@output_stream< cacc48_t > *C[4 1]@t37@{Q2{P{Tinput_stream{1{t{Scint16}}}}}}t37@{Q2{P{Tinput_stream{1{t{Scint16}}}}}}t35@{P{Tinput_stream{1{t{Scacc48_t}}}}}t36@{P{Toutput_stream{1{t{Scacc48_t}}}}}C[4 1]@t5@inputt5@inputt5@inputt6@outputC[4 1]@l0@l0@l0@l0@C[4 1]@l0@l0@l0@l0@C[4 1]@l0@l0@l0@l0@C[4 1]@l0@l0@l0@l1@t281@namespace DoubleStream {
      | template < int NSamples, int ShiftAcc, bool DiscardSample, bool SwapRead > 
      | void FIR_MultiKernel_cincout::
      | filter(input_stream_cint16 * restrict sin1, input_stream_cint16 * restrict sin2, input_stream< cacc48_t > * cin, output_stream< cacc48_t > * cout);
      | }t4@nonee[0 1]@e[0 1]@e[0 1]@e[0 1]@e[0 1]@t132@namespace DoubleStream {
      | template < int NSamples, int ShiftAcc, bool DiscardSample, bool SwapRead > class FIR_MultiKernel_cincout;
      | }t8@implicitC[4 1]@t8@NSamplest8@ShiftAcct13@DiscardSamplet8@SwapReadC[4 1]@t7@nontypet7@nontypet7@nontypet7@nontypeC[4 1]@t3@intt3@intt4@boolt4@boolC[4 1]@nnnnC[4 1]@l1@l1@l1@l1@C[1 1]@t54@FIR_MultiKernel_cincout(cint16 const ( & taps ) [ 4 ])C[1 1]@C[1 1]@t4@tapsC[1 1]@C[1 1]@t23@cint16 const ( &) [ 4 ]C[1 1]@C[1 1]@t20@{R{Q1{C{Scint16}4}}}
      FunctionDecl=|
      | namespace DoubleStream {
      | template < int NSamples, int ShiftAcc, bool DiscardSample, bool SwapRead > 
      | void FIR_MultiKernel_cincout::
      | filter(input_stream_cint16 * restrict sin1, input_stream_cint16 * restrict sin2, input_stream< cacc48_t > * cin, output_stream< cacc48_t > * cout);
      | }
      ClassDeclTypeOptions=|
      | C[1 1]@t132@namespace DoubleStream {
      | template < int NSamples, int ShiftAcc, bool DiscardSample, bool SwapRead > class FIR_MultiKernel_cincout;
      | }
      ClassDecl=|
      | namespace DoubleStream {
      | template < int NSamples, int ShiftAcc, bool DiscardSample, bool SwapRead > class FIR_MultiKernel_cincout;
      | }
  filter5 : ModelComposer/AIE Class Kernel  KernelAllAttrs=|  PortNames={'sin1'; 'sin2'; 'cin'; 'cout'}  PortSerializedTypes={'{Q2{P{Tinput_stream{1{t{Scint16}}}}}}'; '{Q2{P{Tinput_stream{1{t{Scint16}}}}}}'; '{P{Tinput_stream{1{t{Scacc48_t}}}}}'; '{P{Toutput_stream{1{t{Scacc48_t}}}}}'}  PortWindowSizes={0.000000000000000000e+00; 0.000000000000000000e+00; 0.000000000000000000e+00; 0.000000000000000000e+00}  PortWindowMargins={0.000000000000000000e+00; 0.000000000000000000e+00; 0.000000000000000000e+00; 0.000000000000000000e+00}  PortSynchronicities={'auto'; 'auto'; 'auto'; 'auto'}  PortSignalSizes={0.000000000000000000e+00; 0.000000000000000000e+00; 0.000000000000000000e+00; 8.000000000000000000e+00}  ClassTemplateSpecKind=implicit  ClassTemplateParamNames={'NSamples'; 'ShiftAcc'; 'DiscardSample'; 'SwapRead'}  ClassTemplateParamKinds={'nontype'; 'nontype'; 'nontype'; 'nontype'}  ClassTemplateParamTypes={'int'; 'int'; 'bool'; 'bool'}  ClassTemplateParamValues={'512', '15', '0', '0'}  ClassCtorParamNames={'taps'}  ClassCtorParamSerializedTypes={'{R{Q1{C{Scint16}4}}}'}  ClassCtorParamValues={'[-160-111i 248+2878i 1183-239i -21-26i]'}  ClassIndex=1  ClassCtorIndex=1  ClassTabVisible=on  ClassTemplateParamsVisible=on  ClassCtorDeclVisible=on  ClassCtorParamsVisible=on  FunctionTabVisible=on  FunctionDecl=|  PortAttrs={ 'input', 'sin1', 'input_stream_cint16 * restrict', '', '', '', ''; 'input', 'sin2', 'input_stream_cint16 * restrict', '', '', '', ''; 'input', 'cin', 'input_stream< cacc48_t > *', '', '', '', ''; 'output', 'cout', 'output_stream< cacc48_t > *', '', '', '', 'OUTPUT_SIZE' }  PortAttrsEnables={'off', 'off', 'off', 'off', 'off', 'off', 'off';'off', 'off', 'off', 'off', 'off', 'off', 'off';'off', 'off', 'off', 'off', 'off', 'off', 'off';'off', 'off', 'off', 'off', 'off', 'off', 'on'}  SampleTime=-1  ClassDeclTypeOptions=|  ClassDecl=|  ClassTemplateParams={ 'NSamples', 'int', 'BURST_LENGTH'; 'ShiftAcc', 'int', 'SHIFT_ACC'; 'DiscardSample', 'bool', 'FALSE'; 'SwapRead', 'bool', 'FALSE' }  ClassTemplateParamsEnables={'off', 'off', 'on';'off', 'off', 'on';'off', 'off', 'on';'off', 'off', 'on'}  ClassCtorDeclTypeOptions=C[1 1]@t54@FIR_MultiKernel_cincout(cint16 const ( & taps ) [ 4 ])  ClassCtorDecl=FIR_MultiKernel_cincout(cint16 const ( & taps ) [ 4 ])  ClassCtorParams={ 'taps', 'cint16 const ( &) [ 4 ]', 'phi_5' }  KernelHeaderFile=FirDoubleStream.h  KernelClassName=DoubleStream::FIR_MultiKernel_cincout  KernelFunction=filter  KernelSourceFile=FirDoubleStream.cpp  KernelSearchPaths={'$SRC/aie_kernels'}  PreProcOptions={}  CoreRuntimeRatio=0.9  KernelLocSpec=off  ColRowLocation=[0 0]  blockJsonConstraints="{\"type\":\"constraint\",\"constraintType\":\"coreUtilization\",\"sid\":\"2\",\"lhs\":{\"type\":\"runtimeRatio\",\"args\":{\"type\":\"kernel\",\"name\":\"DualStreamSSR_1/Subsystem/filter1\",\"sid\":\"2\"}},\"rhs\":{\"type\":\"evaluable\",\"expr\":\"0.9\",\"value\":0.9},\"equality\":true}"  deprecateConstraints=1
      KernelAllAttrs=|
      | s[12;12;9;9;19;14;21;23;24;21;12;24;26;26;26;27;28;9;21;23;23;23;24;25;14;19;19;29]@FunctionNameDeclFileNamePortNamesPortTypesPortSerializedTypesPortDirectionsPortWindowSizeEnablesPortWindowMarginEnablesPortSynchronicityEnablesPortSignalSizeEnablesFunctionDeclFunctionTemplateSpecKindFunctionTemplateParamNamesFunctionTemplateParamKindsFunctionTemplateParamTypesFunctionTemplateParamValuesFunctionTemplateParamEnablesClassDeclClassTemplateSpecKindClassTemplateParamNamesClassTemplateParamKindsClassTemplateParamTypesClassTemplateParamValuesClassTemplateParamEnablesClassCtorDeclsClassCtorParamNamesClassCtorParamTypesClassCtorParamSerializedTypes[1 1]@C[28 1]@t6@filtert42@../../../aie/aie_kernels/FirDoubleStream.hC[4 1]@t4@sin1t4@sin2t3@cint4@coutC[4 1]@t30@input_stream_cint16 * restrictt30@input_stream_cint16 * restrictt26@input_stream< cacc48_t > *t27@output_stream< cacc48_t > *C[4 1]@t37@{Q2{P{Tinput_stream{1{t{Scint16}}}}}}t37@{Q2{P{Tinput_stream{1{t{Scint16}}}}}}t35@{P{Tinput_stream{1{t{Scacc48_t}}}}}t36@{P{Toutput_stream{1{t{Scacc48_t}}}}}C[4 1]@t5@inputt5@inputt5@inputt6@outputC[4 1]@l0@l0@l0@l0@C[4 1]@l0@l0@l0@l0@C[4 1]@l0@l0@l0@l0@C[4 1]@l0@l0@l0@l1@t281@namespace DoubleStream {
      | template < int NSamples, int ShiftAcc, bool DiscardSample, bool SwapRead > 
      | void FIR_MultiKernel_cincout::
      | filter(input_stream_cint16 * restrict sin1, input_stream_cint16 * restrict sin2, input_stream< cacc48_t > * cin, output_stream< cacc48_t > * cout);
      | }t4@nonee[0 1]@e[0 1]@e[0 1]@e[0 1]@e[0 1]@t132@namespace DoubleStream {
      | template < int NSamples, int ShiftAcc, bool DiscardSample, bool SwapRead > class FIR_MultiKernel_cincout;
      | }t8@implicitC[4 1]@t8@NSamplest8@ShiftAcct13@DiscardSamplet8@SwapReadC[4 1]@t7@nontypet7@nontypet7@nontypet7@nontypeC[4 1]@t3@intt3@intt4@boolt4@boolC[4 1]@nnnnC[4 1]@l1@l1@l1@l1@C[1 1]@t54@FIR_MultiKernel_cincout(cint16 const ( & taps ) [ 4 ])C[1 1]@C[1 1]@t4@tapsC[1 1]@C[1 1]@t23@cint16 const ( &) [ 4 ]C[1 1]@C[1 1]@t20@{R{Q1{C{Scint16}4}}}
      FunctionDecl=|
      | namespace DoubleStream {
      | template < int NSamples, int ShiftAcc, bool DiscardSample, bool SwapRead > 
      | void FIR_MultiKernel_cincout::
      | filter(input_stream_cint16 * restrict sin1, input_stream_cint16 * restrict sin2, input_stream< cacc48_t > * cin, output_stream< cacc48_t > * cout);
      | }
      ClassDeclTypeOptions=|
      | C[1 1]@t132@namespace DoubleStream {
      | template < int NSamples, int ShiftAcc, bool DiscardSample, bool SwapRead > class FIR_MultiKernel_cincout;
      | }
      ClassDecl=|
      | namespace DoubleStream {
      | template < int NSamples, int ShiftAcc, bool DiscardSample, bool SwapRead > class FIR_MultiKernel_cincout;
      | }
  filter50 : ModelComposer/AIE Class Kernel  KernelAllAttrs=|  PortNames={'sin1'; 'sin2'; 'cin'; 'cout'}  PortSerializedTypes={'{Q2{P{Tinput_stream{1{t{Scint16}}}}}}'; '{Q2{P{Tinput_stream{1{t{Scint16}}}}}}'; '{P{Tinput_stream{1{t{Scacc48_t}}}}}'; '{P{Toutput_stream{1{t{Scacc48_t}}}}}'}  PortWindowSizes={0.000000000000000000e+00; 0.000000000000000000e+00; 0.000000000000000000e+00; 0.000000000000000000e+00}  PortWindowMargins={0.000000000000000000e+00; 0.000000000000000000e+00; 0.000000000000000000e+00; 0.000000000000000000e+00}  PortSynchronicities={'auto'; 'auto'; 'auto'; 'auto'}  PortSignalSizes={0.000000000000000000e+00; 0.000000000000000000e+00; 0.000000000000000000e+00; 8.000000000000000000e+00}  ClassTemplateSpecKind=implicit  ClassTemplateParamNames={'NSamples'; 'ShiftAcc'; 'DiscardSample'; 'SwapRead'}  ClassTemplateParamKinds={'nontype'; 'nontype'; 'nontype'; 'nontype'}  ClassTemplateParamTypes={'int'; 'int'; 'bool'; 'bool'}  ClassTemplateParamValues={'512', '15', '1', '0'}  ClassCtorParamNames={'taps'}  ClassCtorParamSerializedTypes={'{R{Q1{C{Scint16}4}}}'}  ClassCtorParamValues={'[-160-111i 248+2878i 1183-239i -21-26i]'}  ClassIndex=1  ClassCtorIndex=1  ClassTabVisible=on  ClassTemplateParamsVisible=on  ClassCtorDeclVisible=on  ClassCtorParamsVisible=on  FunctionTabVisible=on  FunctionDecl=|  PortAttrs={ 'input', 'sin1', 'input_stream_cint16 * restrict', '', '', '', ''; 'input', 'sin2', 'input_stream_cint16 * restrict', '', '', '', ''; 'input', 'cin', 'input_stream< cacc48_t > *', '', '', '', ''; 'output', 'cout', 'output_stream< cacc48_t > *', '', '', '', 'OUTPUT_SIZE' }  PortAttrsEnables={'off', 'off', 'off', 'off', 'off', 'off', 'off';'off', 'off', 'off', 'off', 'off', 'off', 'off';'off', 'off', 'off', 'off', 'off', 'off', 'off';'off', 'off', 'off', 'off', 'off', 'off', 'on'}  SampleTime=-1  ClassDeclTypeOptions=|  ClassDecl=|  ClassTemplateParams={ 'NSamples', 'int', 'BURST_LENGTH'; 'ShiftAcc', 'int', 'SHIFT_ACC'; 'DiscardSample', 'bool', 'TRUE'; 'SwapRead', 'bool', 'FALSE' }  ClassTemplateParamsEnables={'off', 'off', 'on';'off', 'off', 'on';'off', 'off', 'on';'off', 'off', 'on'}  ClassCtorDeclTypeOptions=C[1 1]@t54@FIR_MultiKernel_cincout(cint16 const ( & taps ) [ 4 ])  ClassCtorDecl=FIR_MultiKernel_cincout(cint16 const ( & taps ) [ 4 ])  ClassCtorParams={ 'taps', 'cint16 const ( &) [ 4 ]', 'phi_5' }  KernelHeaderFile=FirDoubleStream.h  KernelClassName=DoubleStream::FIR_MultiKernel_cincout  KernelFunction=filter  KernelSourceFile=FirDoubleStream.cpp  KernelSearchPaths={'$SRC/aie_kernels'}  PreProcOptions={}  CoreRuntimeRatio=0.9  KernelLocSpec=off  ColRowLocation=[0 0]  blockJsonConstraints="{\"type\":\"constraint\",\"constraintType\":\"coreUtilization\",\"sid\":\"60\",\"lhs\":{\"type\":\"runtimeRatio\",\"args\":{\"type\":\"kernel\",\"name\":\"DualStreamSSR_1/Subsystem/filter41\",\"sid\":\"60\"}},\"rhs\":{\"type\":\"evaluable\",\"expr\":\"0.9\",\"value\":0.9},\"equality\":true}"  deprecateConstraints=1
      KernelAllAttrs=|
      | s[12;12;9;9;19;14;21;23;24;21;12;24;26;26;26;27;28;9;21;23;23;23;24;25;14;19;19;29]@FunctionNameDeclFileNamePortNamesPortTypesPortSerializedTypesPortDirectionsPortWindowSizeEnablesPortWindowMarginEnablesPortSynchronicityEnablesPortSignalSizeEnablesFunctionDeclFunctionTemplateSpecKindFunctionTemplateParamNamesFunctionTemplateParamKindsFunctionTemplateParamTypesFunctionTemplateParamValuesFunctionTemplateParamEnablesClassDeclClassTemplateSpecKindClassTemplateParamNamesClassTemplateParamKindsClassTemplateParamTypesClassTemplateParamValuesClassTemplateParamEnablesClassCtorDeclsClassCtorParamNamesClassCtorParamTypesClassCtorParamSerializedTypes[1 1]@C[28 1]@t6@filtert42@../../../aie/aie_kernels/FirDoubleStream.hC[4 1]@t4@sin1t4@sin2t3@cint4@coutC[4 1]@t30@input_stream_cint16 * restrictt30@input_stream_cint16 * restrictt26@input_stream< cacc48_t > *t27@output_stream< cacc48_t > *C[4 1]@t37@{Q2{P{Tinput_stream{1{t{Scint16}}}}}}t37@{Q2{P{Tinput_stream{1{t{Scint16}}}}}}t35@{P{Tinput_stream{1{t{Scacc48_t}}}}}t36@{P{Toutput_stream{1{t{Scacc48_t}}}}}C[4 1]@t5@inputt5@inputt5@inputt6@outputC[4 1]@l0@l0@l0@l0@C[4 1]@l0@l0@l0@l0@C[4 1]@l0@l0@l0@l0@C[4 1]@l0@l0@l0@l1@t281@namespace DoubleStream {
      | template < int NSamples, int ShiftAcc, bool DiscardSample, bool SwapRead > 
      | void FIR_MultiKernel_cincout::
      | filter(input_stream_cint16 * restrict sin1, input_stream_cint16 * restrict sin2, input_stream< cacc48_t > * cin, output_stream< cacc48_t > * cout);
      | }t4@nonee[0 1]@e[0 1]@e[0 1]@e[0 1]@e[0 1]@t132@namespace DoubleStream {
      | template < int NSamples, int ShiftAcc, bool DiscardSample, bool SwapRead > class FIR_MultiKernel_cincout;
      | }t8@implicitC[4 1]@t8@NSamplest8@ShiftAcct13@DiscardSamplet8@SwapReadC[4 1]@t7@nontypet7@nontypet7@nontypet7@nontypeC[4 1]@t3@intt3@intt4@boolt4@boolC[4 1]@nnnnC[4 1]@l1@l1@l1@l1@C[1 1]@t54@FIR_MultiKernel_cincout(cint16 const ( & taps ) [ 4 ])C[1 1]@C[1 1]@t4@tapsC[1 1]@C[1 1]@t23@cint16 const ( &) [ 4 ]C[1 1]@C[1 1]@t20@{R{Q1{C{Scint16}4}}}
      FunctionDecl=|
      | namespace DoubleStream {
      | template < int NSamples, int ShiftAcc, bool DiscardSample, bool SwapRead > 
      | void FIR_MultiKernel_cincout::
      | filter(input_stream_cint16 * restrict sin1, input_stream_cint16 * restrict sin2, input_stream< cacc48_t > * cin, output_stream< cacc48_t > * cout);
      | }
      ClassDeclTypeOptions=|
      | C[1 1]@t132@namespace DoubleStream {
      | template < int NSamples, int ShiftAcc, bool DiscardSample, bool SwapRead > class FIR_MultiKernel_cincout;
      | }
      ClassDecl=|
      | namespace DoubleStream {
      | template < int NSamples, int ShiftAcc, bool DiscardSample, bool SwapRead > class FIR_MultiKernel_cincout;
      | }
  filter51 : ModelComposer/AIE Class Kernel  KernelAllAttrs=|  PortNames={'sin1'; 'sin2'; 'cin'; 'cout'}  PortSerializedTypes={'{Q2{P{Tinput_stream{1{t{Scint16}}}}}}'; '{Q2{P{Tinput_stream{1{t{Scint16}}}}}}'; '{P{Tinput_stream{1{t{Scacc48_t}}}}}'; '{P{Toutput_stream{1{t{Scacc48_t}}}}}'}  PortWindowSizes={0.000000000000000000e+00; 0.000000000000000000e+00; 0.000000000000000000e+00; 0.000000000000000000e+00}  PortWindowMargins={0.000000000000000000e+00; 0.000000000000000000e+00; 0.000000000000000000e+00; 0.000000000000000000e+00}  PortSynchronicities={'auto'; 'auto'; 'auto'; 'auto'}  PortSignalSizes={0.000000000000000000e+00; 0.000000000000000000e+00; 0.000000000000000000e+00; 8.000000000000000000e+00}  ClassTemplateSpecKind=implicit  ClassTemplateParamNames={'NSamples'; 'ShiftAcc'; 'DiscardSample'; 'SwapRead'}  ClassTemplateParamKinds={'nontype'; 'nontype'; 'nontype'; 'nontype'}  ClassTemplateParamTypes={'int'; 'int'; 'bool'; 'bool'}  ClassTemplateParamValues={'512', '15', '1', '0'}  ClassCtorParamNames={'taps'}  ClassCtorParamSerializedTypes={'{R{Q1{C{Scint16}4}}}'}  ClassCtorParamValues={'[146-91i 4086+5221i 237-54i -83-21i]'}  ClassIndex=1  ClassCtorIndex=1  ClassTabVisible=on  ClassTemplateParamsVisible=on  ClassCtorDeclVisible=on  ClassCtorParamsVisible=on  FunctionTabVisible=on  FunctionDecl=|  PortAttrs={ 'input', 'sin1', 'input_stream_cint16 * restrict', '', '', '', ''; 'input', 'sin2', 'input_stream_cint16 * restrict', '', '', '', ''; 'input', 'cin', 'input_stream< cacc48_t > *', '', '', '', ''; 'output', 'cout', 'output_stream< cacc48_t > *', '', '', '', 'OUTPUT_SIZE' }  PortAttrsEnables={'off', 'off', 'off', 'off', 'off', 'off', 'off';'off', 'off', 'off', 'off', 'off', 'off', 'off';'off', 'off', 'off', 'off', 'off', 'off', 'off';'off', 'off', 'off', 'off', 'off', 'off', 'on'}  SampleTime=-1  ClassDeclTypeOptions=|  ClassDecl=|  ClassTemplateParams={ 'NSamples', 'int', 'BURST_LENGTH'; 'ShiftAcc', 'int', 'SHIFT_ACC'; 'DiscardSample', 'bool', 'TRUE'; 'SwapRead', 'bool', 'FALSE' }  ClassTemplateParamsEnables={'off', 'off', 'on';'off', 'off', 'on';'off', 'off', 'on';'off', 'off', 'on'}  ClassCtorDeclTypeOptions=C[1 1]@t54@FIR_MultiKernel_cincout(cint16 const ( & taps ) [ 4 ])  ClassCtorDecl=FIR_MultiKernel_cincout(cint16 const ( & taps ) [ 4 ])  ClassCtorParams={ 'taps', 'cint16 const ( &) [ 4 ]', 'phi_6' }  KernelHeaderFile=FirDoubleStream.h  KernelClassName=DoubleStream::FIR_MultiKernel_cincout  KernelFunction=filter  KernelSourceFile=FirDoubleStream.cpp  KernelSearchPaths={'$SRC/aie_kernels'}  PreProcOptions={}  CoreRuntimeRatio=0.9  KernelLocSpec=off  ColRowLocation=[0 0]  blockJsonConstraints="{\"type\":\"constraint\",\"constraintType\":\"coreUtilization\",\"sid\":\"60\",\"lhs\":{\"type\":\"runtimeRatio\",\"args\":{\"type\":\"kernel\",\"name\":\"DualStreamSSR_1/Subsystem/filter41\",\"sid\":\"60\"}},\"rhs\":{\"type\":\"evaluable\",\"expr\":\"0.9\",\"value\":0.9},\"equality\":true}"  deprecateConstraints=1
      KernelAllAttrs=|
      | s[12;12;9;9;19;14;21;23;24;21;12;24;26;26;26;27;28;9;21;23;23;23;24;25;14;19;19;29]@FunctionNameDeclFileNamePortNamesPortTypesPortSerializedTypesPortDirectionsPortWindowSizeEnablesPortWindowMarginEnablesPortSynchronicityEnablesPortSignalSizeEnablesFunctionDeclFunctionTemplateSpecKindFunctionTemplateParamNamesFunctionTemplateParamKindsFunctionTemplateParamTypesFunctionTemplateParamValuesFunctionTemplateParamEnablesClassDeclClassTemplateSpecKindClassTemplateParamNamesClassTemplateParamKindsClassTemplateParamTypesClassTemplateParamValuesClassTemplateParamEnablesClassCtorDeclsClassCtorParamNamesClassCtorParamTypesClassCtorParamSerializedTypes[1 1]@C[28 1]@t6@filtert42@../../../aie/aie_kernels/FirDoubleStream.hC[4 1]@t4@sin1t4@sin2t3@cint4@coutC[4 1]@t30@input_stream_cint16 * restrictt30@input_stream_cint16 * restrictt26@input_stream< cacc48_t > *t27@output_stream< cacc48_t > *C[4 1]@t37@{Q2{P{Tinput_stream{1{t{Scint16}}}}}}t37@{Q2{P{Tinput_stream{1{t{Scint16}}}}}}t35@{P{Tinput_stream{1{t{Scacc48_t}}}}}t36@{P{Toutput_stream{1{t{Scacc48_t}}}}}C[4 1]@t5@inputt5@inputt5@inputt6@outputC[4 1]@l0@l0@l0@l0@C[4 1]@l0@l0@l0@l0@C[4 1]@l0@l0@l0@l0@C[4 1]@l0@l0@l0@l1@t281@namespace DoubleStream {
      | template < int NSamples, int ShiftAcc, bool DiscardSample, bool SwapRead > 
      | void FIR_MultiKernel_cincout::
      | filter(input_stream_cint16 * restrict sin1, input_stream_cint16 * restrict sin2, input_stream< cacc48_t > * cin, output_stream< cacc48_t > * cout);
      | }t4@nonee[0 1]@e[0 1]@e[0 1]@e[0 1]@e[0 1]@t132@namespace DoubleStream {
      | template < int NSamples, int ShiftAcc, bool DiscardSample, bool SwapRead > class FIR_MultiKernel_cincout;
      | }t8@implicitC[4 1]@t8@NSamplest8@ShiftAcct13@DiscardSamplet8@SwapReadC[4 1]@t7@nontypet7@nontypet7@nontypet7@nontypeC[4 1]@t3@intt3@intt4@boolt4@boolC[4 1]@nnnnC[4 1]@l1@l1@l1@l1@C[1 1]@t54@FIR_MultiKernel_cincout(cint16 const ( & taps ) [ 4 ])C[1 1]@C[1 1]@t4@tapsC[1 1]@C[1 1]@t23@cint16 const ( &) [ 4 ]C[1 1]@C[1 1]@t20@{R{Q1{C{Scint16}4}}}
      FunctionDecl=|
      | namespace DoubleStream {
      | template < int NSamples, int ShiftAcc, bool DiscardSample, bool SwapRead > 
      | void FIR_MultiKernel_cincout::
      | filter(input_stream_cint16 * restrict sin1, input_stream_cint16 * restrict sin2, input_stream< cacc48_t > * cin, output_stream< cacc48_t > * cout);
      | }
      ClassDeclTypeOptions=|
      | C[1 1]@t132@namespace DoubleStream {
      | template < int NSamples, int ShiftAcc, bool DiscardSample, bool SwapRead > class FIR_MultiKernel_cincout;
      | }
      ClassDecl=|
      | namespace DoubleStream {
      | template < int NSamples, int ShiftAcc, bool DiscardSample, bool SwapRead > class FIR_MultiKernel_cincout;
      | }
  filter52 : ModelComposer/AIE Class Kernel  KernelAllAttrs=|  PortNames={'sin1'; 'sin2'; 'cin'; 'cout'}  PortSerializedTypes={'{Q2{P{Tinput_stream{1{t{Scint16}}}}}}'; '{Q2{P{Tinput_stream{1{t{Scint16}}}}}}'; '{P{Tinput_stream{1{t{Scacc48_t}}}}}'; '{P{Toutput_stream{1{t{Scacc48_t}}}}}'}  PortWindowSizes={0.000000000000000000e+00; 0.000000000000000000e+00; 0.000000000000000000e+00; 0.000000000000000000e+00}  PortWindowMargins={0.000000000000000000e+00; 0.000000000000000000e+00; 0.000000000000000000e+00; 0.000000000000000000e+00}  PortSynchronicities={'auto'; 'auto'; 'auto'; 'auto'}  PortSignalSizes={0.000000000000000000e+00; 0.000000000000000000e+00; 0.000000000000000000e+00; 8.000000000000000000e+00}  ClassTemplateSpecKind=implicit  ClassTemplateParamNames={'NSamples'; 'ShiftAcc'; 'DiscardSample'; 'SwapRead'}  ClassTemplateParamKinds={'nontype'; 'nontype'; 'nontype'; 'nontype'}  ClassTemplateParamTypes={'int'; 'int'; 'bool'; 'bool'}  ClassTemplateParamValues={'512', '15', '1', '0'}  ClassCtorParamNames={'taps'}  ClassCtorParamSerializedTypes={'{R{Q1{C{Scint16}4}}}'}  ClassCtorParamValues={'[342-439i 8773+2748i 102+525i -54+21i]'}  ClassIndex=1  ClassCtorIndex=1  ClassTabVisible=on  ClassTemplateParamsVisible=on  ClassCtorDeclVisible=on  ClassCtorParamsVisible=on  FunctionTabVisible=on  FunctionDecl=|  PortAttrs={ 'input', 'sin1', 'input_stream_cint16 * restrict', '', '', '', ''; 'input', 'sin2', 'input_stream_cint16 * restrict', '', '', '', ''; 'input', 'cin', 'input_stream< cacc48_t > *', '', '', '', ''; 'output', 'cout', 'output_stream< cacc48_t > *', '', '', '', 'OUTPUT_SIZE' }  PortAttrsEnables={'off', 'off', 'off', 'off', 'off', 'off', 'off';'off', 'off', 'off', 'off', 'off', 'off', 'off';'off', 'off', 'off', 'off', 'off', 'off', 'off';'off', 'off', 'off', 'off', 'off', 'off', 'on'}  SampleTime=-1  ClassDeclTypeOptions=|  ClassDecl=|  ClassTemplateParams={ 'NSamples', 'int', 'BURST_LENGTH'; 'ShiftAcc', 'int', 'SHIFT_ACC'; 'DiscardSample', 'bool', 'TRUE'; 'SwapRead', 'bool', 'FALSE' }  ClassTemplateParamsEnables={'off', 'off', 'on';'off', 'off', 'on';'off', 'off', 'on';'off', 'off', 'on'}  ClassCtorDeclTypeOptions=C[1 1]@t54@FIR_MultiKernel_cincout(cint16 const ( & taps ) [ 4 ])  ClassCtorDecl=FIR_MultiKernel_cincout(cint16 const ( & taps ) [ 4 ])  ClassCtorParams={ 'taps', 'cint16 const ( &) [ 4 ]', 'phi_7' }  KernelHeaderFile=FirDoubleStream.h  KernelClassName=DoubleStream::FIR_MultiKernel_cincout  KernelFunction=filter  KernelSourceFile=FirDoubleStream.cpp  KernelSearchPaths={'$SRC/aie_kernels'}  PreProcOptions={}  CoreRuntimeRatio=0.9  KernelLocSpec=off  ColRowLocation=[0 0]  blockJsonConstraints="{\"type\":\"constraint\",\"constraintType\":\"coreUtilization\",\"sid\":\"60\",\"lhs\":{\"type\":\"runtimeRatio\",\"args\":{\"type\":\"kernel\",\"name\":\"DualStreamSSR_1/Subsystem/filter41\",\"sid\":\"60\"}},\"rhs\":{\"type\":\"evaluable\",\"expr\":\"0.9\",\"value\":0.9},\"equality\":true}"  deprecateConstraints=1
